simulink library "DQN_Lib (conflicted copy 2023-11-25 155310)"  (R2023b)
settings: Solver=VariableStepAuto  StartTime=0.0  StopTime=10.0  RelTol=1e-3
undefined symbols (not defined in the file): FreqRad, HrmOrd, Init, La, N, R, Ra, TimeStep, Ts, Ts_dqn, Ws
libraries: $bdroot x4, spsMeanVariableFrequencyLib x4, eeTransforms x3, spsabctodq0Lib x2, spsAlphaBetaZerotodq0Lib x1
(part 4 of 8)

== matlab function DQN_Lib (conflicted copy 2023-11-25 155310)/DQn (Full)10 ==
  data: Zdc output size=3; Xdc input size=3; Xdp input; Xdn input; Xdz input; Xqp input; Xqn input; Xqz input; Ydc input size=3; Ydp input; Ydn input; Ydz input; Yqp input; Yqn input; Yqz input; Zdp output; Zdn output; Zdz output; Zqp output; Zqn output; N parameter; Zqz output
function [Zdc,Zdp,Zdn,Zdz,Zqp,Zqn,Zqz]  = MultDQN(Xdc, Xdp, Xdn, Xdz, Xqp, Xqn, Xqz, Ydc, Ydp, Ydn, Ydz, Yqp, Yqn, Yqz, N)

    Zdc = zeros(3,1);
    a = -0.5+0.866i;
    a2 = -0.5-0.866i;
    T = [1 1 1;1 a a2;1 a2 a];

    Xdp = [Xdp; zeros(N-numel(Xdp),1)];
    Ydp = [Ydp; zeros(N-numel(Ydp),1)];
    Xqp = [Xqp; zeros(N-numel(Xqp),1)];
    Yqp = [Yqp; zeros(N-numel(Yqp),1)];
      
    Xdn = [Xdn; zeros(N-numel(Xdn),1)];
    Ydn = [Ydn; zeros(N-numel(Ydn),1)];
    Xqn = [Xqn; zeros(N-numel(Xqn),1)];
    Yqn = [Yqn; zeros(N-numel(Yqn),1)];
    
    Xdz = [Xdz; zeros(N-numel(Xdz),1)];
    Ydz = [Ydz; zeros(N-numel(Ydz),1)];
    Xqz = [Xqz; zeros(N-numel(Xqz),1)];
    Yqz = [Yqz; zeros(N-numel(Yqz),1)];
    
    Zdp = zeros(2*N,1);
    Zdn = zeros(2*N,1);
    Zqp = zeros(2*N,1);
    Zqn = zeros(2*N,1);
    Zdz = zeros(2*N,1);
    Zqz = zeros(2*N,1);
         
    Zdc = Xdc.*Ydc;
    
   
    for h = 1 : 2*N
        if(h<=N)

            Zdc = Zdc + 0.5*(Xdp(h)*Ydp(h)+Xqp(h)*Yqp(h));
            Zdc = Zdc + 0.5*(Xdn(h)*Ydn(h)+Xqn(h)*Yqn(h));
            Zdc = Zdc + 0.5*(Xdz(h)*Ydz(h)+Xqz(h)*Yqz(h));


            Ymp = sqrt(Ydp(h)^2+Yqp(h)^2);
            Yap = atan2(Yqp(h),+Ydp(h));  


            Ymn = sqrt(Ydn(h)^2+Yqn(h)^2);
            Yan = atan2(Yqn(h),-Ydn(h));  

            Xmz = sqrt(Xdz(h)^2+Xqz(h)^2);
            Xaz = atan2(Xqz(h),+Xdz(h));  
            Ymz = sqrt(Ydz(h)^2+Yqz(h)^2);
            Yaz = atan2(Yqz(h),+Ydz(h));  

            
            Xmp = sqrt(Xdp(h)^2+Xqp(h)^2);
            Xap = atan2(Xqp(h),+Xdp(h));  
            if(Xmp~=0)
            Zdz(2*h) = Zdz(2*h) + 0.5*Xmp*Ymn*sin(Xap+Yan);
            Zqz(2*h) = Zqz(2*h) - 0.5*Xmp*Ymn*cos(Xap+Yan);
            Zdc = Zdc + 0.5*Xmp*Ymn*[cos(Xap-Yan); cos(Xap-Yan-4*pi/3); cos(Xap-Yan+4*pi/3)];
            Zdc = Zdc + 0.5*Xmp*Ymz*[cos(Xap-Yaz); cos(Xap-Yaz+4*pi/3); cos(Xap-Yaz-4*pi/3)];
            end

            Xmn = sqrt(Xdn(h)^2+Xqn(h)^2);
            Xan = atan2(Xqn(h),-Xdn(h));  
            if(Xmn~=0)
            Zdz(2*h) = Zdz(2*h) + 0.5*Xmn*Ymp*sin(Xan+Yap);
            Zqz(2*h) = Zqz(2*h) - 0.5*Xmn*Ymp*cos(Xan+Yap);
            Zdc = Zdc + 0.5*Xmn*Ymp*[cos(Xan-Yap); cos(Xan-Yap+4*pi/3); cos(Xan-Yap-4*pi/3)];
            Zdc = Zdc + 0.5*Xmn*Ymz*[cos(Xan-Yaz); cos(Xan-Yaz-4*pi/3); cos(Xan-Yaz+4*pi/3)];
            end
            
            if(Xmz~=0)
            Zdc = Zdc + 0.5*Xmz*Ymp*[cos(Xaz-Yap); cos(Xaz-Yap-4*pi/3); cos(Xaz-Yap+4*pi/3)];
            Zdc = Zdc + 0.5*Xmz*Ymn*[cos(Xaz-Yan); cos(Xaz-Yan+4*pi/3); cos(Xaz-Yan-4*pi/3)];
            end

            if(all(Xdc == Xdc(1)) && all(Ydc == Ydc(1)))
                Zdp(h) = Zdp(h) + Xdc(1)*Ydp(h)+Xdp(h)*Ydc(1);     
                Zqp(h) = Zqp(h) + Xdc(1)*Yqp(h)+Xqp(h)*Ydc(1);  
                Zdn(h) = Zdn(h) + Xdc(1)*Ydn(h)+Xdn(h)*Ydc(1);
                Zqn(h) = Zqn(h) + Xdc(1)*Yqn(h)+Xqn(h)*Ydc(1);
                Zdz(h) = Zdz(h) + Xdc(1)*Ydz(h)+Xdz(h)*Ydc(1);     
                Zqz(h) = Zqz(h) + Xdc(1)*Yqz(h)+Xqz(h)*Ydc(1); 
            else
                %%%%%%%%%%%%%%%%% POSITIVE (Ydc*Xp) %%%%%%%%%%%%%%%%%%%
                if(Xmp ~= 0)
%                     V_ABC = [Ydc(1)*Xmp*(cos(Xap)       +1i*sin(Xap));
%                              Ydc(2)*Xmp*(cos(Xap-2*pi/3)+1i*sin(Xap-2*pi/3));
%                              Ydc(3)*Xmp*(cos(Xap+2*pi/3)+1i*sin(Xap+2*pi/3))];
%                     V_012 = T*V_ABC/3;
                    
                    V_012 = T*[Ydc(1)*Xmp*(cos(Xap)       +1i*sin(Xap));
                               Ydc(2)*Xmp*(cos(Xap-2*pi/3)+1i*sin(Xap-2*pi/3));
                               Ydc(3)*Xmp*(cos(Xap+2*pi/3)+1i*sin(Xap+2*pi/3))]/3;

                    Zdz(h) = Zdz(h) + real(V_012(1)); Zqz(h) = Zqz(h) + imag(V_012(1));
                    Zdp(h) = Zdp(h) + real(V_012(2)); Zqp(h) = Zqp(h) + imag(V_012(2));
                    Zdn(h) = Zdn(h) - real(V_012(3)); Zqn(h) = Zqn(h) + imag(V_012(3));
                end
                %%%%%%%%%%%%%%%%% POSITIVE (Xdc*Yp) %%%%%%%%%%%%%%%%%%%
                if(Ymp ~= 0)
%                 V_ABC = [Xdc(1)*Ymp*(cos(Yap)       +1i*sin(Yap));
%                          Xdc(2)*Ymp*(cos(Yap-2*pi/3)+1i*sin(Yap-2*pi/3));
%                          Xdc(3)*Ymp*(cos(Yap+2*pi/3)+1i*sin(Yap+2*pi/3))];
%                 V_012 = T*V_ABC/3;
                
                V_012 = T*[Xdc(1)*Ymp*(cos(Yap)       +1i*sin(Yap));
                         Xdc(2)*Ymp*(cos(Yap-2*pi/3)+1i*sin(Yap-2*pi/3));
                         Xdc(3)*Ymp*(cos(Yap+2*pi/3)+1i*sin(Yap+2*pi/3))]/3;

                Zdz(h) = Zdz(h) + real(V_012(1)); Zqz(h) = Zqz(h) + imag(V_012(1));
                Zdp(h) = Zdp(h) + real(V_012(2)); Zqp(h) = Zqp(h) + imag(V_012(2));
                Zdn(h) = Zdn(h) - real(V_012(3)); Zqn(h) = Zqn(h) + imag(V_012(3));
                end
                %%%%%%%%%%%%%%%%% NEGATIVE (Ydc*Xn) %%%%%%%%%%%%%%%%%%%
                if(Xmn ~= 0)
                    V_012 = T*[Ydc(1)*Xmn*(cos(Xan)       +1i*sin(Xan));
                             Ydc(2)*Xmn*(cos(Xan+2*pi/3)+1i*sin(Xan+2*pi/3));
                             Ydc(3)*Xmn*(cos(Xan-2*pi/3)+1i*sin(Xan-2*pi/3))]/3;
                    

                    Zdz(h) = Zdz(h) + real(V_012(1)); Zqz(h) = Zqz(h) + imag(V_012(1));
                    Zdp(h) = Zdp(h) + real(V_012(2)); Zqp(h) = Zqp(h) + imag(V_012(2));
                    Zdn(h) = Zdn(h) - real(V_012(3)); Zqn(h) = Zqn(h) + imag(V_012(3));
                end
                %%%%%%%%%%%%%%%%% NEGATIVE (Xdc*Yn) %%%%%%%%%%%%%%%%%%%
                if(Ymn ~= 0)
                    V_012 = T*[Xdc(1)*Ymn*(cos(Yan)       +1i*sin(Yan));
                             Xdc(2)*Ymn*(cos(Yan+2*pi/3)+1i*sin(Yan+2*pi/3));
                             Xdc(3)*Ymn*(cos(Yan-2*pi/3)+1i*sin(Yan-2*pi/3))]/3;

                    Zdz(h) = Zdz(h) + real(V_012(1)); Zqz(h) = Zqz(h) + imag(V_012(1));
                    Zdp(h) = Zdp(h) + real(V_012(2)); Zqp(h) = Zqp(h) + imag(V_012(2));
                    Zdn(h) = Zdn(h) - real(V_012(3)); Zqn(h) = Zqn(h) + imag(V_012(3));
                end
                %%%%%%%%%%%%%%%%%%%%%%%%%%%%%%%%%%%%%%%%%%%%%%%%%%%%%%
                if(Xmz ~= 0)
                    V_012 = T*[Ydc(1)*Xmz*(cos(Xaz)+1i*sin(Xaz));
                               Ydc(2)*Xmz*(cos(Xaz)+1i*sin(Xaz));
                               Ydc(3)*Xmz*(cos(Xaz)+1i*sin(Xaz))]/3;
                    

                    Zdz(h) = Zdz(h) + real(V_012(1)); Zqz(h) = Zqz(h) + imag(V_012(1));
                    Zdp(h) = Zdp(h) + real(V_012(2)); Zqp(h) = Zqp(h) + imag(V_012(2));
                    Zdn(h) = Zdn(h) - real(V_012(3)); Zqn(h) = Zqn(h) + imag(V_012(3));
                end
                %%%%%%%%%%%%%%%%%%%%%%%%%%%%%%%%%%%%%%%%%%%%%%%%%%%%%%

                if(Ymz ~= 0)
                    V_012 = T*[Xdc(1)*Ymz*(cos(Yaz)+1i*sin(Yaz));
                             Xdc(2)*Ymz*(cos(Yaz)+1i*sin(Yaz));
                             Xdc(3)*Ymz*(cos(Yaz)+1i*sin(Yaz))]/3;
                    
                    Zdz(h) = Zdz(h) + real(V_012(1)); Zqz(h) = Zqz(h) + imag(V_012(1));
                    Zdp(h) = Zdp(h) + real(V_012(2)); Zqp(h) = Zqp(h) + imag(V_012(2));
                    Zdn(h) = Zdn(h) - real(V_012(3)); Zqn(h) = Zqn(h) + imag(V_012(3));
                end
            end
            
%%%%%%%%%%%%%%%%%%%%%% h<=N ODD %%%%%%%%%%%%%%%%%%%%%%%%%%%%%%%%%%%%%%%%%
            if(mod(h,2)==1) 
                %%%%%%%%%%%%%%%%% D3p (3ph+) %%%%%%%%%%%%%%%%%%%%%%%

                %&%%%%%%%%%%%%%%%%%%%%%%%%%% PP + NN %%%%%%%%%%%%%%%%%%%%%%%%%%%
                for i = 1 : h - 1
                   Zdp(h) = Zdp(h) - 0.5*(Xdn(i)*Yqn(h-i) + Xqn(i)*Ydn(h-i));                    
                   Zdn(h) = Zdn(h) - 0.5*(Xdp(i)*Yqp(h-i) + Xqp(i)*Ydp(h-i)); 
                   Zqp(h) = Zqp(h) - 0.5*(Xdn(i)*Ydn(h-i) - Xqn(i)*Yqn(h-i));                
                   Zqn(h) = Zqn(h) - 0.5*(Xdp(i)*Ydp(h-i) - Xqp(i)*Yqp(h-i)); 
                end

                for i = 1 : N - h
                    Zdz(h) = Zdz(h) + 0.5*(-Xdp(i)*Yqp(i+h) + Xqp(i)*Ydp(i+h) + Xdp(i+h)*Yqp(i) - Xqp(i+h)*Ydp(i) + Xdn(i)*Yqn(i+h) - Xqn(i)*Ydn(i+h) - Xdn(i+h)*Yqn(i) + Xqn(i+h)*Ydn(i));  
                    Zqz(h) = Zqz(h) + 0.5*(+Xdp(i)*Ydp(i+h) + Xqp(i)*Yqp(i+h) + Xdp(i+h)*Ydp(i) + Xqp(i+h)*Yqp(i) + Xdn(i)*Ydn(i+h) + Xqn(i)*Yqn(i+h) + Xdn(i+h)*Ydn(i) + Xqn(i+h)*Yqn(i));    
                end
                %&%%%%%%%%%%%%%%%%%%%%%%%%%% PP + NN %%%%%%%%%%%%%%%%%%%%%%%%%%%

                for k = 1 : (N + mod(N+1,2) - h)/2
                    i = 2*k-1;
                    j = i+h;

                    Zdz(h)  = Zdz(h)  + 0.5*(-Xdz(i)*Yqz(j) + Xqz(i)*Ydz(j) + Xdz(j)*Yqz(i) - Xqz(j)*Ydz(i));
                    Zqz(h)  = Zqz(h)  + 0.5*(+Xdz(i)*Ydz(j) + Xqz(i)*Yqz(j) + Xdz(j)*Ydz(i) + Xqz(j)*Yqz(i)); 

                    Zdp(h) = Zdp(h) + 0.5*(-Xdp(i)*Yqn(j) - Xqp(i)*Ydn(j) - Xdn(j)*Yqp(i) - Xqn(j)*Ydp(i)); 
                    Zdp(h) = Zdp(h) + 0.5*(-Xdz(i)*Yqp(j) + Xqz(i)*Ydp(j) + Xdp(j)*Yqz(i) - Xqp(j)*Ydz(i));    
                    Zdp(h) = Zdp(h) + 0.5*(+Xdn(i)*Yqz(j) + Xqn(i)*Ydz(j) + Xdz(j)*Yqn(i) + Xqz(j)*Ydn(i));
                    
                    Zqp(h) = Zqp(h) + 0.5*(-Xdp(i)*Ydn(j) + Xqp(i)*Yqn(j) - Xdn(j)*Ydp(i) + Xqn(j)*Yqp(i));  
                    Zqp(h) = Zqp(h) + 0.5*(+Xdz(i)*Ydp(j) + Xqz(i)*Yqp(j) + Xdp(j)*Ydz(i) + Xqp(j)*Yqz(i));     
                    Zqp(h) = Zqp(h) + 0.5*(-Xdn(i)*Ydz(j) + Xqn(i)*Yqz(j) - Xdz(j)*Ydn(i) + Xqz(j)*Yqn(i));

                    Zdn(h) = Zdn(h) + 0.5*(+Xdp(i)*Yqz(j) - Xqp(i)*Ydz(j) - Xdz(j)*Yqp(i) + Xqz(j)*Ydp(i));             
                    Zdn(h) = Zdn(h) + 0.5*(+Xdz(i)*Yqn(j) + Xqz(i)*Ydn(j) + Xdn(j)*Yqz(i) + Xqn(j)*Ydz(i));
                    Zdn(h) = Zdn(h) + 0.5*(-Xdn(i)*Yqp(j) - Xqn(i)*Ydp(j) - Xdp(j)*Yqn(i) - Xqp(j)*Ydn(i)); 

                    Zqn(h) = Zqn(h) + 0.5*(+Xdp(i)*Ydz(j) + Xqp(i)*Yqz(j) + Xdz(j)*Ydp(i) + Xqz(j)*Yqp(i)); 
                    Zqn(h) = Zqn(h) + 0.5*(-Xdz(i)*Ydn(j) + Xqz(i)*Yqn(j) - Xdn(j)*Ydz(i) + Xqn(j)*Yqz(i)); 
                    Zqn(h) = Zqn(h) + 0.5*(-Xdn(i)*Ydp(j) + Xqn(i)*Yqp(j) - Xdp(j)*Ydn(i) + Xqp(j)*Yqn(i));  
                end

                for k = 1 : (N + mod(N,2) - h - 1)/2
                    i = 2*k;
                    j = i+h;
                    
                    Zdz(h) = Zdz(h)   + 0.5*(-Xdz(i)*Yqz(j) + Xqz(i)*Ydz(j) + Xdz(j)*Yqz(i) - Xqz(j)*Ydz(i));
                    Zqz(h) = Zqz(h)   + 0.5*(+Xdz(i)*Ydz(j) + Xqz(i)*Yqz(j) + Xdz(j)*Ydz(i) + Xqz(j)*Yqz(i)); 

                    Zdp(h) = Zdp(h) + 0.5*(-Xdp(i)*Yqn(j) - Xqp(i)*Ydn(j) - Xdn(j)*Yqp(i) - Xqn(j)*Ydp(i)); 
                    Zqp(h) = Zqp(h) + 0.5*(-Xdp(i)*Ydn(j) + Xqp(i)*Yqn(j) - Xdn(j)*Ydp(i) + Xqn(j)*Yqp(i));  
                    Zdn(h) = Zdn(h) + 0.5*(-Xdn(i)*Yqp(j) - Xqn(i)*Ydp(j) - Xdp(j)*Yqn(i) - Xqp(j)*Ydn(i)); 
                    Zqn(h) = Zqn(h) + 0.5*(-Xdn(i)*Ydp(j) + Xqn(i)*Yqp(j) - Xdp(j)*Ydn(i) + Xqp(j)*Yqn(i));                                          

                    Zdp(h) = Zdp(h) + 0.5*(-Xdz(i)*Yqp(j) + Xqz(i)*Ydp(j) + Xdp(j)*Yqz(i) - Xqp(j)*Ydz(i));
                    Zqp(h) = Zqp(h) + 0.5*(+Xdz(i)*Ydp(j) + Xqz(i)*Yqp(j) + Xdp(j)*Ydz(i) + Xqp(j)*Yqz(i));                     
                    Zdn(h) = Zdn(h) + 0.5*(+Xdp(i)*Yqz(j) - Xqp(i)*Ydz(j) - Xdz(j)*Yqp(i) + Xqz(j)*Ydp(i));
                    Zqn(h) = Zqn(h) + 0.5*(+Xdp(i)*Ydz(j) + Xqp(i)*Yqz(j) + Xdz(j)*Ydp(i) + Xqz(j)*Yqp(i));   

                    Zdp(h) = Zdp(h) + 0.5*(+Xdn(i)*Yqz(j) + Xqn(i)*Ydz(j) + Xdz(j)*Yqn(i) + Xqz(j)*Ydn(i));
                    Zqp(h) = Zqp(h) + 0.5*(-Xdn(i)*Ydz(j) + Xqn(i)*Yqz(j) - Xdz(j)*Ydn(i) + Xqz(j)*Yqn(i));                
                    Zdn(h) = Zdn(h) + 0.5*(+Xdz(i)*Yqn(j) + Xqz(i)*Ydn(j) + Xdn(j)*Yqz(i) + Xqn(j)*Ydz(i));
                    Zqn(h) = Zqn(h) + 0.5*(-Xdz(i)*Ydn(j) + Xqz(i)*Yqn(j) - Xdn(j)*Ydz(i) + Xqn(j)*Yqz(i)); 

                end

                for k = (h-1)/2:-1:1
                    i = k;
                    j = h-i;  
                    
                    Zdz(h) = Zdz(h) + 0.5*(+Xdp(i)*Yqn(j)-Xqp(i)*Ydn(j)-Xdn(j)*Yqp(i)+Xqn(j)*Ydp(i));
                    Zqz(h) = Zqz(h) + 0.5*(+Xdp(i)*Ydn(j)+Xqp(i)*Yqn(j)+Xdn(j)*Ydp(i)+Xqn(j)*Yqp(i));
                    Zdz(h) = Zdz(h) + 0.5*(+Xdp(j)*Yqn(i)-Xqp(j)*Ydn(i)-Xdn(i)*Yqp(j)+Xqn(i)*Ydp(j));
                    Zqz(h) = Zqz(h) + 0.5*(+Xdp(j)*Ydn(i)+Xqp(j)*Yqn(i)+Xdn(i)*Ydp(j)+Xqn(i)*Yqp(j)); 
                    Zdz(h) = Zdz(h) + 0.5*(+Xdz(i)*Yqz(j)+Xqz(i)*Ydz(j)+Xdz(j)*Yqz(i)+Xqz(j)*Ydz(i));
                    Zqz(h) = Zqz(h) + 0.5*(-Xdz(i)*Ydz(j)+Xqz(i)*Yqz(j)-Xdz(j)*Ydz(i)+Xqz(j)*Yqz(i));    
                        
                        
                    Zdp(h) = Zdp(h) + 0.5*(+Xdz(i)*Yqp(j)+Xqz(i)*Ydp(j)+Xdz(j)*Yqp(i)+Xqz(j)*Ydp(i));
                    Zqp(h) = Zqp(h) + 0.5*(-Xdz(i)*Ydp(j)+Xqz(i)*Yqp(j)-Xdz(j)*Ydp(i)+Xqz(j)*Yqp(i));
                    Zdp(h) = Zdp(h) + 0.5*(+Xdp(i)*Yqz(j)+Xqp(i)*Ydz(j)+Xdp(j)*Yqz(i)+Xqp(j)*Ydz(i));
                    Zqp(h) = Zqp(h) + 0.5*(-Xdp(i)*Ydz(j)+Xqp(i)*Yqz(j)-Xdp(j)*Ydz(i)+Xqp(j)*Yqz(i)); 
                    
                              
                    Zdn(h) = Zdn(h) + 0.5*(+Xdn(i)*Yqz(j)-Xqn(i)*Ydz(j)+Xdn(j)*Yqz(i)-Xqn(j)*Ydz(i));
                    Zqn(h) = Zqn(h) + 0.5*(+Xdn(i)*Ydz(j)+Xqn(i)*Yqz(j)+Xdn(j)*Ydz(i)+Xqn(j)*Yqz(i)); 
                    Zdn(h) = Zdn(h) + 0.5*(-Xdz(i)*Yqn(j)+Xqz(i)*Ydn(j)-Xdz(j)*Yqn(i)+Xqz(j)*Ydn(i));
                    Zqn(h) = Zqn(h) + 0.5*(+Xdz(i)*Ydn(j)+Xqz(i)*Yqn(j)+Xdz(j)*Ydn(i)+Xqz(j)*Yqn(i)); 
                end
%%%%%%%%%%%%%%%%%%%%%% h<=N EVEN %%%%%%%%%%%%%%%%%%%%%%%%%%%%%%%%%%%%%%%%%           
            else 
               
                Zdp(h) = Zdp(h) + 0.5*(-Xdn(h/2)*Yqn(h/2)-Xqn(h/2)*Ydn(h/2));   
                Zqp(h) = Zqp(h) + 0.5*(-Xdn(h/2)*Ydn(h/2)+Xqn(h/2)*Yqn(h/2)); 
                Zdn(h) = Zdn(h) + 0.5*(-Xdp(h/2)*Yqp(h/2)-Xqp(h/2)*Ydp(h/2));   
                Zqn(h) = Zqn(h) + 0.5*(-Xdp(h/2)*Ydp(h/2)+Xqp(h/2)*Yqp(h/2));   

                Zdz(h)  = Zdz(h)  + 0.5*(+Xdz(h/2)*Yqz(h/2)+Xqz(h/2)*Ydz(h/2));
                Zqz(h)  = Zqz(h)  + 0.5*(-Xdz(h/2)*Ydz(h/2)+Xqz(h/2)*Yqz(h/2));

                Zdp(h) = Zdp(h) + 0.5*(+Xdz(h/2)*Yqp(h/2)+Xqz(h/2)*Ydp(h/2)+Xdp(h/2)*Yqz(h/2)+Xqp(h/2)*Ydz(h/2));   
                Zqp(h) = Zqp(h) + 0.5*(-Xdz(h/2)*Ydp(h/2)+Xqz(h/2)*Yqp(h/2)-Xdp(h/2)*Ydz(h/2)+Xqp(h/2)*Yqz(h/2)); 
                Zdn(h) = Zdn(h) + 0.5*(+Xdn(h/2)*Yqz(h/2)-Xqn(h/2)*Ydz(h/2)-Xdz(h/2)*Yqn(h/2)+Xqz(h/2)*Ydn(h/2));   
                Zqn(h) = Zqn(h) + 0.5*(+Xdn(h/2)*Ydz(h/2)+Xqn(h/2)*Yqz(h/2)+Xdz(h/2)*Ydn(h/2)+Xqz(h/2)*Yqn(h/2));    
                
                for k = 1:N-h
                    i = k;
                    j = h+i;
                
                    Zdz(h) = Zdz(h)   + 0.5*(+Xdp(j)*Yqp(i) - Xqp(j)*Ydp(i) - Xdp(i)*Yqp(j) + Xqp(i)*Ydp(j));
                    Zqz(h) = Zqz(h)   + 0.5*(+Xdp(j)*Ydp(i) + Xqp(j)*Yqp(i) + Xdp(i)*Ydp(j) + Xqp(i)*Yqp(j));                                           
                    Zdz(h) = Zdz(h)   + 0.5*(+Xdn(i)*Yqn(j) - Xqn(i)*Ydn(j) - Xdn(j)*Yqn(i) + Xqn(j)*Ydn(i));
                    Zqz(h) = Zqz(h)   + 0.5*(+Xdn(i)*Ydn(j) + Xqn(i)*Yqn(j) + Xdn(j)*Ydn(i) + Xqn(j)*Yqn(i));  
                    Zdz(h) = Zdz(h)   + 0.5*(-Xdz(i)*Yqz(j) + Xqz(i)*Ydz(j) + Xdz(j)*Yqz(i) - Xqz(j)*Ydz(i));
                    Zqz(h) = Zqz(h)   + 0.5*(+Xdz(i)*Ydz(j) + Xqz(i)*Yqz(j) + Xdz(j)*Ydz(i) + Xqz(j)*Yqz(i)); 
                                       
                    Zdp(h) = Zdp(h) + 0.5*(-Xdp(i)*Yqn(j) - Xqp(i)*Ydn(j) - Xdn(j)*Yqp(i) - Xqn(j)*Ydp(i)); 
                    Zqp(h) = Zqp(h) + 0.5*(-Xdp(i)*Ydn(j) + Xqp(i)*Yqn(j) - Xdn(j)*Ydp(i) + Xqn(j)*Yqp(i)); 
                    Zdn(h) = Zdn(h) + 0.5*(-Xdn(i)*Yqp(j) - Xqn(i)*Ydp(j) - Xdp(j)*Yqn(i) - Xqp(j)*Ydn(i)); 
                    Zqn(h) = Zqn(h) + 0.5*(-Xdn(i)*Ydp(j) + Xqn(i)*Yqp(j) - Xdp(j)*Ydn(i) + Xqp(j)*Yqn(i)); 
                        
                    Zdp(h) = Zdp(h) + 0.5*(+Xdp(j)*Yqz(i) - Xqp(j)*Ydz(i) - Xdz(i)*Yqp(j) + Xqz(i)*Ydp(j));
                    Zqp(h) = Zqp(h) + 0.5*(+Xdp(j)*Ydz(i) + Xqp(j)*Yqz(i) + Xdz(i)*Ydp(j) + Xqz(i)*Yqp(j)); 
                    Zdn(h) = Zdn(h) + 0.5*(+Xdp(i)*Yqz(j) - Xqp(i)*Ydz(j) - Xdz(j)*Yqp(i) + Xqz(j)*Ydp(i));
                    Zqn(h) = Zqn(h) + 0.5*(+Xdp(i)*Ydz(j) + Xqp(i)*Yqz(j) + Xdz(j)*Ydp(i) + Xqz(j)*Yqp(i)); 
                    
                    Zdp(h) = Zdp(h) + 0.5*(+Xdn(i)*Yqz(j) + Xqn(i)*Ydz(j) + Xdz(j)*Yqn(i) + Xqz(j)*Ydn(i));
                    Zqp(h) = Zqp(h) + 0.5*(-Xdn(i)*Ydz(j) + Xqn(i)*Yqz(j) - Xdz(j)*Ydn(i) + Xqz(j)*Yqn(i)); 
                    Zdn(h) = Zdn(h) + 0.5*(+Xdn(j)*Yqz(i) + Xqn(j)*Ydz(i) + Xdz(i)*Yqn(j) + Xqz(i)*Ydn(j));
                    Zqn(h) = Zqn(h) + 0.5*(-Xdn(j)*Ydz(i) + Xqn(j)*Yqz(i) - Xdz(i)*Ydn(j) + Xqz(i)*Yqn(j)); 
                end

                for k = h/2-1:-1:1
                    i = k;
                    j = h-i;   

                    Zdz(h) = Zdz(h)   + 0.5*(+Xdp(i)*Yqn(j) - Xqp(i)*Ydn(j) + Xdp(j)*Yqn(i) - Xqp(j)*Ydn(i));
                    Zdz(h) = Zdz(h)   + 0.5*(-Xdn(i)*Yqp(j) + Xqn(i)*Ydp(j) - Xdn(j)*Yqp(i) + Xqn(j)*Ydp(i));      
                    Zdz(h) = Zdz(h)   + 0.5*(+Xdz(i)*Yqz(j) + Xqz(i)*Ydz(j) + Xdz(j)*Yqz(i) + Xqz(j)*Ydz(i));
                    
                    Zqz(h) = Zqz(h)   + 0.5*(+Xdp(i)*Ydn(j) + Xqp(i)*Yqn(j) + Xdp(j)*Ydn(i) + Xqp(j)*Yqn(i)); 
                    Zqz(h) = Zqz(h)   + 0.5*(+Xdn(i)*Ydp(j) + Xqn(i)*Yqp(j) + Xdn(j)*Ydp(i) + Xqn(j)*Yqp(i));
                    Zqz(h) = Zqz(h)   + 0.5*(-Xdz(i)*Ydz(j) + Xqz(i)*Yqz(j) - Xdz(j)*Ydz(i) + Xqz(j)*Yqz(i)); 
                    
                    Zdp(h) = Zdp(h) + 0.5*(+Xdp(i)*Yqz(j) + Xqp(i)*Ydz(j) + Xdp(j)*Yqz(i) + Xqp(j)*Ydz(i)); 
                    Zdp(h) = Zdp(h) + 0.5*(-Xdn(i)*Yqn(j) - Xqn(i)*Ydn(j) - Xdn(j)*Yqn(i) - Xqn(j)*Ydn(i)); 
                    Zdp(h) = Zdp(h) + 0.5*(+Xdz(i)*Yqp(j) + Xqz(i)*Ydp(j) + Xdz(j)*Yqp(i) + Xqz(j)*Ydp(i));
                    
                    Zqp(h) = Zqp(h) + 0.5*(-Xdp(i)*Ydz(j) + Xqp(i)*Yqz(j) - Xdp(j)*Ydz(i) + Xqp(j)*Yqz(i)); 
                    Zqp(h) = Zqp(h) + 0.5*(-Xdn(i)*Ydn(j) + Xqn(i)*Yqn(j) - Xdn(j)*Ydn(i) + Xqn(j)*Yqn(i));
                    Zqp(h) = Zqp(h) + 0.5*(-Xdz(i)*Ydp(j) + Xqz(i)*Yqp(j) - Xdz(j)*Ydp(i) + Xqz(j)*Yqp(i));  
                    
                    Zdn(h) = Zdn(h) + 0.5*(-Xdp(i)*Yqp(j) - Xqp(i)*Ydp(j) - Xdp(j)*Yqp(i) - Xqp(j)*Ydp(i));
                    Zdn(h) = Zdn(h) + 0.5*(+Xdn(i)*Yqz(j) - Xqn(i)*Ydz(j) + Xdn(j)*Yqz(i) - Xqn(j)*Ydz(i));
                    Zdn(h) = Zdn(h) + 0.5*(-Xdz(i)*Yqn(j) + Xqz(i)*Ydn(j) - Xdz(j)*Yqn(i) + Xqz(j)*Ydn(i));
                    
                    Zqn(h) = Zqn(h) + 0.5*(-Xdp(i)*Ydp(j) + Xqp(i)*Yqp(j) - Xdp(j)*Ydp(i) + Xqp(j)*Yqp(i));  
                    Zqn(h) = Zqn(h) + 0.5*(+Xdn(i)*Ydz(j) + Xqn(i)*Yqz(j) + Xdn(j)*Ydz(i) + Xqn(j)*Yqz(i));
                    Zqn(h) = Zqn(h) + 0.5*(+Xdz(i)*Ydn(j) + Xqz(i)*Yqn(j) + Xdz(j)*Ydn(i) + Xqz(j)*Yqn(i)); 
                end
            end
%%%%%%%%%%%%%%%%%%%%%%%%%%%% h>N  %%%%%%%%%%%%%%%%%%%%%%%%%%%%%%%%%%%%%%%%% 
        else %h>N
            
            
            %%%%%%%%%%%%%%%%%%%%%%%%%%% PP + NN %%%%%%%%%%%%%%%%%%%%%%%%%%%
            for i = h-N : N
                Zdp(h) = Zdp(h) - 0.5*(Xdn(i)*Yqn(h-i) + Xqn(i)*Ydn(h-i));                
                Zdn(h) = Zdn(h) - 0.5*(Xdp(i)*Yqp(h-i) + Xqp(i)*Ydp(h-i));                     
                Zqp(h) = Zqp(h) - 0.5*(Xdn(i)*Ydn(h-i) - Xqn(i)*Yqn(h-i));                      
                Zqn(h) = Zqn(h) - 0.5*(Xdp(i)*Ydp(h-i) - Xqp(i)*Yqp(h-i));   
            end
            %%%%%%%%%%%%%%%%%%%%%%%%%%% PP + NN %%%%%%%%%%%%%%%%%%%%%%%%%%%

            if(mod(h,2)==1) %%%%%%%%%%% h>N ODD %%%%%%%%%%%%%%%%%%%

                for k = (h-1)/2:-1:h-N
                    i = k;
                    j = h-i;
                    
                    Zdz(h) = Zdz(h) + 0.5*(+Xdp(i)*Yqn(j)-Xqp(i)*Ydn(j)-Xdn(j)*Yqp(i)+Xqn(j)*Ydp(i));                  
                    Zdz(h) = Zdz(h) + 0.5*(+Xdp(j)*Yqn(i)-Xqp(j)*Ydn(i)-Xdn(i)*Yqp(j)+Xqn(i)*Ydp(j));
                    Zdz(h) = Zdz(h) + 0.5*(+Xdz(i)*Yqz(j)+Xqz(i)*Ydz(j)+Xdz(j)*Yqz(i)+Xqz(j)*Ydz(i));
                    
                    Zqz(h) = Zqz(h) + 0.5*(-Xdz(i)*Ydz(j)+Xqz(i)*Yqz(j)-Xdz(j)*Ydz(i)+Xqz(j)*Yqz(i));
                    Zqz(h) = Zqz(h) + 0.5*(+Xdp(i)*Ydn(j)+Xqp(i)*Yqn(j)+Xdn(j)*Ydp(i)+Xqn(j)*Yqp(i));
                    Zqz(h) = Zqz(h) + 0.5*(+Xdp(j)*Ydn(i)+Xqp(j)*Yqn(i)+Xdn(i)*Ydp(j)+Xqn(i)*Yqp(j));  
                    
                    Zdp(h) = Zdp(h) + 0.5*(+Xdp(i)*Yqz(j)+Xqp(i)*Ydz(j)+Xdp(j)*Yqz(i)+Xqp(j)*Ydz(i));
                    Zdp(h) = Zdp(h) + 0.5*(+Xdz(i)*Yqp(j)+Xqz(i)*Ydp(j)+Xdz(j)*Yqp(i)+Xqz(j)*Ydp(i));
                    
                    Zqp(h) = Zqp(h) + 0.5*(-Xdp(i)*Ydz(j)+Xqp(i)*Yqz(j)-Xdp(j)*Ydz(i)+Xqp(j)*Yqz(i)); 
                    Zqp(h) = Zqp(h) + 0.5*(-Xdz(i)*Ydp(j)+Xqz(i)*Yqp(j)-Xdz(j)*Ydp(i)+Xqz(j)*Yqp(i));     
                                       
                    Zdn(h) = Zdn(h) + 0.5*(+Xdn(i)*Yqz(j)-Xqn(i)*Ydz(j)+Xdn(j)*Yqz(i)-Xqn(j)*Ydz(i));
                    Zdn(h) = Zdn(h) + 0.5*(-Xdz(i)*Yqn(j)+Xqz(i)*Ydn(j)-Xdz(j)*Yqn(i)+Xqz(j)*Ydn(i));
                    
                    Zqn(h) = Zqn(h) + 0.5*(+Xdn(i)*Ydz(j)+Xqn(i)*Yqz(j)+Xdn(j)*Ydz(i)+Xqn(j)*Yqz(i));
                    Zqn(h) = Zqn(h) + 0.5*(+Xdz(i)*Ydn(j)+Xqz(i)*Yqn(j)+Xdz(j)*Ydn(i)+Xqz(j)*Yqn(i));    

                end

            else %%%%%%%%%%% h>N EVEN %%%%%%%%%%%%%%%%%%%

                Zdz(h)  = Zdz(h)  + 0.5*(+Xdz(h/2)*Yqz(h/2)+Xqz(h/2)*Ydz(h/2));
                Zqz(h)  = Zqz(h)  + 0.5*(-Xdz(h/2)*Ydz(h/2)+Xqz(h/2)*Yqz(h/2));
                
                Zdp(h) = 0.5*(-Xdn(h/2)*Yqn(h/2)-Xqn(h/2)*Ydn(h/2));          
                Zdp(h) = Zdp(h) + 0.5*(+Xdp(h/2)*Yqz(h/2)+Xqp(h/2)*Ydz(h/2));                
                Zdp(h) = Zdp(h) + 0.5*(+Xdz(h/2)*Yqp(h/2)+Xqz(h/2)*Ydp(h/2));    
                
                Zqp(h) = 0.5*(-Xdn(h/2)*Ydn(h/2)+Xqn(h/2)*Yqn(h/2));             
                Zqp(h) = Zqp(h) + 0.5*(-Xdp(h/2)*Ydz(h/2)+Xqp(h/2)*Yqz(h/2));        
                Zqp(h) = Zqp(h) + 0.5*(-Xdz(h/2)*Ydp(h/2)+Xqz(h/2)*Yqp(h/2)); 
                
                Zdn(h) = 0.5*(-Xdp(h/2)*Yqp(h/2)-Xqp(h/2)*Ydp(h/2)); 
                Zdn(h) = Zdn(h) + 0.5*(+Xdn(h/2)*Yqz(h/2)-Xqn(h/2)*Ydz(h/2));
                Zdn(h) = Zdn(h) + 0.5*(-Xdz(h/2)*Yqn(h/2)+Xqz(h/2)*Ydn(h/2));
                               
                Zqn(h) = 0.5*(-Xdp(h/2)*Ydp(h/2)+Xqp(h/2)*Yqp(h/2)); 
                Zqn(h) = Zqn(h) + 0.5*(+Xdn(h/2)*Ydz(h/2)+Xqn(h/2)*Yqz(h/2));        
                Zqn(h) = Zqn(h) + 0.5*(+Xdz(h/2)*Ydn(h/2)+Xqz(h/2)*Yqn(h/2)); 

                for i = (h+2)/2:N
                    j = h-i;
                    Zdz(h)  = Zdz(h)  + 0.5*(+Xdp(i)*Yqn(j)-Xqp(i)*Ydn(j)+Xdp(j)*Yqn(i)-Xqp(j)*Ydn(i));
                    Zdz(h)  = Zdz(h)  + 0.5*(-Xdn(i)*Yqp(j)+Xqn(i)*Ydp(j)-Xdn(j)*Yqp(i)+Xqn(j)*Ydp(i));
                    Zdz(h)  = Zdz(h)  + 0.5*(+Xdz(i)*Yqz(j)+Xqz(i)*Ydz(j)+Xdz(j)*Yqz(i)+Xqz(j)*Ydz(i));
                    
                    Zqz(h)  = Zqz(h)  + 0.5*(+Xdp(i)*Ydn(j)+Xqp(i)*Yqn(j)+Xdp(j)*Ydn(i)+Xqp(j)*Yqn(i));                      
                    Zqz(h)  = Zqz(h)  + 0.5*(+Xdn(i)*Ydp(j)+Xqn(i)*Yqp(j)+Xdn(j)*Ydp(i)+Xqn(j)*Yqp(i));  
                    Zqz(h)  = Zqz(h)  + 0.5*(-Xdz(i)*Ydz(j)+Xqz(i)*Yqz(j)-Xdz(j)*Ydz(i)+Xqz(j)*Yqz(i));
                    
                    Zdp(h) = Zdp(h) + 0.5*(+Xdp(i)*Yqz(j)+Xqp(i)*Ydz(j)+Xdp(j)*Yqz(i)+Xqp(j)*Ydz(i));  
                    Zdp(h) = Zdp(h) + 0.5*(-Xdn(i)*Yqn(j)-Xqn(i)*Ydn(j)-Xdn(j)*Yqn(i)-Xqn(j)*Ydn(i));             
                    Zdp(h) = Zdp(h) + 0.5*(+Xdz(i)*Yqp(j)+Xqz(i)*Ydp(j)+Xdz(j)*Yqp(i)+Xqz(j)*Ydp(i));           
                    
                    Zqp(h) = Zqp(h) + 0.5*(-Xdp(i)*Ydz(j)+Xqp(i)*Yqz(j)-Xdp(j)*Ydz(i)+Xqp(j)*Yqz(i));
                    Zqp(h) = Zqp(h) + 0.5*(-Xdn(i)*Ydn(j)+Xqn(i)*Yqn(j)-Xdn(j)*Ydn(i)+Xqn(j)*Yqn(i));    
                    Zqp(h) = Zqp(h) + 0.5*(-Xdz(i)*Ydp(j)+Xqz(i)*Yqp(j)-Xdz(j)*Ydp(i)+Xqz(j)*Yqp(i));   
                    
                    Zdn(h) = Zdn(h) + 0.5*(-Xdp(i)*Yqp(j)-Xqp(i)*Ydp(j)-Xdp(j)*Yqp(i)-Xqp(j)*Ydp(i));
                    Zdn(h) = Zdn(h) + 0.5*(+Xdn(i)*Yqz(j)-Xqn(i)*Ydz(j)+Xdn(j)*Yqz(i)-Xqn(j)*Ydz(i));
                    Zdn(h) = Zdn(h) + 0.5*(-Xdz(i)*Yqn(j)+Xqz(i)*Ydn(j)-Xdz(j)*Yqn(i)+Xqz(j)*Ydn(i));              
                    
                    Zqn(h) = Zqn(h) + 0.5*(-Xdp(i)*Ydp(j)+Xqp(i)*Yqp(j)-Xdp(j)*Ydp(i)+Xqp(j)*Yqp(i));
                    Zqn(h) = Zqn(h) + 0.5*(+Xdn(i)*Ydz(j)+Xqn(i)*Yqz(j)+Xdn(j)*Ydz(i)+Xqn(j)*Yqz(i)); 
                    Zqn(h) = Zqn(h) + 0.5*(+Xdz(i)*Ydn(j)+Xqz(i)*Yqn(j)+Xdz(j)*Ydn(i)+Xqz(j)*Yqn(i));  
                end
            end
        end  
    end
end
  

% function [Zdc,Zdp,Zdn,Zdz,Zqp,Zqn,Zqz]  = MultDQN(Xdc, Xdp, Xdn, Xdz, Xqp, Xqn, Xqz, Ydc, Ydp, Ydn, Ydz, Yqp, Yqn, Yqz, N)
% 
%     Zdc = zeros(3,1);
%     a = -0.5+0.866i;
%     a2 = -0.5-0.866i;
%     T = [1 1 1;1 a a2;1 a2 a];
% 
%     Xdp = [Xdp; zeros(N-numel(Xdp),1)];
%     Ydp = [Ydp; zeros(N-numel(Ydp),1)];
%     Xqp = [Xqp; zeros(N-numel(Xqp),1)];
%     Yqp = [Yqp; zeros(N-numel(Yqp),1)];
%       
%     Xdn = [Xdn; zeros(N-numel(Xdn),1)];
%     Ydn = [Ydn; zeros(N-numel(Ydn),1)];
%     Xqn = [Xqn; zeros(N-numel(Xqn),1)];
%     Yqn = [Yqn; zeros(N-numel(Yqn),1)];
%     
%     Xdz = [Xdz; zeros(N-numel(Xdz),1)];
%     Ydz = [Ydz; zeros(N-numel(Ydz),1)];
%     Xqz = [Xqz; zeros(N-numel(Xqz),1)];
%     Yqz = [Yqz; zeros(N-numel(Yqz),1)];
%        
%     Zdp = zeros(1,2*N);
%     Zdn = zeros(1,2*N);
%     Zqp = zeros(1,2*N);
%     Zqn = zeros(1,2*N);
%     Zdz = zeros(1,2*N);
%     Zqz = zeros(1,2*N);
%    
%     Zdc = Xdc.*Ydc;
%     
%     
%     for h = 1 : N 
% %         Zdc = Zdc + 0.5*(Xdp(h)*Ydp(h)+Xqp(h)*Yqp(h));
% %         Zdc = Zdc + 0.5*(Xdn(h)*Ydn(h)+Xqn(h)*Yqn(h));
% %         Zdc = Zdc + 0.5*(Xdz(h)*Ydz(h)+Xqz(h)*Yqz(h));
% 
%         Xmp = sqrt(Xdp(h)^2+Xqp(h)^2);
%         Xap = atan2(Xqp(h),+Xdp(h));  
%         Ymp = sqrt(Ydp(h)^2+Yqp(h)^2);
%         Yap = atan2(Yqp(h),+Ydp(h));  
% 
%         Xmn = sqrt(Xdn(h)^2+Xqn(h)^2);
%         Xan = atan2(Xqn(h),-Xdn(h));  
%         Ymn = sqrt(Ydn(h)^2+Yqn(h)^2);
%         Yan = atan2(Yqn(h),-Ydn(h));  
% 
%         Xmz = sqrt(Xdz(h)^2+Xqz(h)^2);
%         Xaz = atan2(Xqz(h),+Xdz(h));  
%         Ymz = sqrt(Ydz(h)^2+Yqz(h)^2);
%         Yaz = atan2(Yqz(h),+Ydz(h));  
% 
%         Zdz(2*h) = Zdz(2*h) + 0.5*Xmp*Ymn*sin(Xap+Yan);
%         Zqz(2*h) = Zqz(2*h) - 0.5*Xmp*Ymn*cos(Xap+Yan);
% 
%         Zdz(2*h) = Zdz(2*h) + 0.5*Xmn*Ymp*sin(Xan+Yap);
%         Zqz(2*h) = Zqz(2*h) - 0.5*Xmn*Ymp*cos(Xan+Yap);
% 
% %         Zdc = Zdc + 0.5*Xmp*Ymn*[cos(Xap-Yan) cos(Xap-Yan-4*pi/3) cos(Xap-Yan+4*pi/3)];
% %         Zdc = Zdc + 0.5*Xmn*Ymp*[cos(Xan-Yap) cos(Xan-Yap+4*pi/3) cos(Xan-Yap-4*pi/3)];
% %         Zdc = Zdc + 0.5*Xmz*Ymp*[cos(Xaz-Yap) cos(Xaz-Yap-4*pi/3) cos(Xaz-Yap+4*pi/3)];
% %         Zdc = Zdc + 0.5*Xmp*Ymz*[cos(Xap-Yaz) cos(Xap-Yaz+4*pi/3) cos(Xap-Yaz-4*pi/3)];
% %         Zdc = Zdc + 0.5*Xmn*Ymz*[cos(Xan-Yaz) cos(Xan-Yaz-4*pi/3) cos(Xan-Yaz+4*pi/3)];
% %         Zdc = Zdc + 0.5*Xmz*Ymn*[cos(Xaz-Yan) cos(Xaz-Yan+4*pi/3) cos(Xaz-Yan-4*pi/3)];
% 
%         if(all(Xdc == Xdc(1)) && all(Ydc == Ydc(1)))
%             Zdp(h) = Zdp(h) + Xdc(1)*Ydp(h)+Xdp(h)*Ydc(1);     
%             Zqp(h) = Zqp(h) + Xdc(1)*Yqp(h)+Xqp(h)*Ydc(1);  
%             Zdn(h) = Zdn(h) + Xdc(1)*Ydn(h)+Xdn(h)*Ydc(1);
%             Zqn(h) = Zqn(h) + Xdc(1)*Yqn(h)+Xqn(h)*Ydc(1);
%             Zdz(h) = Zdz(h) + Xdc(1)*Ydz(h)+Xdz(h)*Ydc(1);     
%             Zqz(h) = Zqz(h) + Xdc(1)*Yqz(h)+Xqz(h)*Ydc(1); 
%         else
%             %%%%%%%%%%%%%%%%% POSITIVE (Ydc*Xp) %%%%%%%%%%%%%%%%%%%
%             if(Xmp ~= 0)
%                 V_ABC = [Ydc(1)*Xmp*(cos(Xap)       +1i*sin(Xap));
%                          Ydc(2)*Xmp*(cos(Xap-2*pi/3)+1i*sin(Xap-2*pi/3));
%                          Ydc(3)*Xmp*(cos(Xap+2*pi/3)+1i*sin(Xap+2*pi/3))];
%                 V_012 = T*V_ABC/3;
% 
%                 Zdz(h) = Zdz(h) + real(V_012(1)); Zqz(h) = Zqz(h) + imag(V_012(1));
%                 Zdp(h) = Zdp(h) + real(V_012(2)); Zqp(h) = Zqp(h) + imag(V_012(2));
%                 Zdn(h) = Zdn(h) - real(V_012(3)); Zqn(h) = Zqn(h) + imag(V_012(3));
%             end
%             %%%%%%%%%%%%%%%%% POSITIVE (Xdc*Yp) %%%%%%%%%%%%%%%%%%%
%             if(Ymp ~= 0)
%             V_ABC = [Xdc(1)*Ymp*(cos(Yap)       +1i*sin(Yap));
%                      Xdc(2)*Ymp*(cos(Yap-2*pi/3)+1i*sin(Yap-2*pi/3));
%                      Xdc(3)*Ymp*(cos(Yap+2*pi/3)+1i*sin(Yap+2*pi/3))];
%             V_012 = T*V_ABC/3;
% 
%             Zdz(h) = Zdz(h) + real(V_012(1)); Zqz(h) = Zqz(h) + imag(V_012(1));
%             Zdp(h) = Zdp(h) + real(V_012(2)); Zqp(h) = Zqp(h) + imag(V_012(2));
%             Zdn(h) = Zdn(h) - real(V_012(3)); Zqn(h) = Zqn(h) + imag(V_012(3));
%             end
%             %%%%%%%%%%%%%%%%% NEGATIVE (Ydc*Xn) %%%%%%%%%%%%%%%%%%%
%             if(Xmn ~= 0)
%                 V_ABC = [Ydc(1)*Xmn*(cos(Xan)       +1i*sin(Xan));
%                          Ydc(2)*Xmn*(cos(Xan+2*pi/3)+1i*sin(Xan+2*pi/3));
%                          Ydc(3)*Xmn*(cos(Xan-2*pi/3)+1i*sin(Xan-2*pi/3))];
%                 V_012 = T*V_ABC/3;
% 
%                 Zdz(h) = Zdz(h) + real(V_012(1)); Zqz(h) = Zqz(h) + imag(V_012(1));
%                 Zdp(h) = Zdp(h) + real(V_012(2)); Zqp(h) = Zqp(h) + imag(V_012(2));
%                 Zdn(h) = Zdn(h) - real(V_012(3)); Zqn(h) = Zqn(h) + imag(V_012(3));
%             end
%             %%%%%%%%%%%%%%%%% NEGATIVE (Xdc*Yn) %%%%%%%%%%%%%%%%%%%
%             if(Ymn ~= 0)
%             V_ABC = [Xdc(1)*Ymn*(cos(Yan)       +1i*sin(Yan));
%                      Xdc(2)*Ymn*(cos(Yan+2*pi/3)+1i*sin(Yan+2*pi/3));
%                      Xdc(3)*Ymn*(cos(Yan-2*pi/3)+1i*sin(Yan-2*pi/3))];
%             V_012 = T*V_ABC/3;
% 
%             Zdz(h) = Zdz(h) + real(V_012(1)); Zqz(h) = Zqz(h) + imag(V_012(1));
%             Zdp(h) = Zdp(h) + real(V_012(2)); Zqp(h) = Zqp(h) + imag(V_012(2));
%             Zdn(h) = Zdn(h) - real(V_012(3)); Zqn(h) = Zqn(h) + imag(V_012(3));
%             end
%             %%%%%%%%%%%%%%%%%%%%%%%%%%%%%%%%%%%%%%%%%%%%%%%%%%%%%%
%             if(Xmz ~= 0)
%                 V_ABC = [Ydc(1)*Xmz*(cos(Xaz)+1i*sin(Xaz));
%                          Ydc(2)*Xmz*(cos(Xaz)+1i*sin(Xaz));
%                          Ydc(3)*Xmz*(cos(Xaz)+1i*sin(Xaz))];
%                 V_012 = T*V_ABC/3;
% 
%                 Zdz(h) = Zdz(h) + real(V_012(1)); Zqz(h) = Zqz(h) + imag(V_012(1));
%                 Zdp(h) = Zdp(h) + real(V_012(2)); Zqp(h) = Zqp(h) + imag(V_012(2));
%                 Zdn(h) = Zdn(h) - real(V_012(3)); Zqn(h) = Zqn(h) + imag(V_012(3));
%             end
%             %%%%%%%%%%%%%%%%%%%%%%%%%%%%%%%%%%%%%%%%%%%%%%%%%%%%%%
% 
%             if(Ymz ~= 0)
%                 V_ABC = [Xdc(1)*Ymz*(cos(Yaz)+1i*sin(Yaz));
%                          Xdc(2)*Ymz*(cos(Yaz)+1i*sin(Yaz));
%                          Xdc(3)*Ymz*(cos(Yaz)+1i*sin(Yaz))];
%                 V_012 = T*V_ABC/3;
%                 Zdz(h) = Zdz(h) + real(V_012(1)); Zqz(h) = Zqz(h) + imag(V_012(1));
%                 Zdp(h) = Zdp(h) + real(V_012(2)); Zqp(h) = Zqp(h) + imag(V_012(2));
%                 Zdn(h) = Zdn(h) - real(V_012(3)); Zqn(h) = Zqn(h) + imag(V_012(3));
%             end
%         end
%     end
% %     
% %     
% %    
% %     for h = 1 : 2*N
% %         if(h<=N)
% % 
% % %%%%%%%%%%%%%%%%%%%%%% h<=N ODD %%%%%%%%%%%%%%%%%%%%%%%%%%%%%%%%%%%%%%%%%
% %             if(mod(h,2)==1) 
% %                 %%%%%%%%%%%%%%%%% D3p (3ph+) %%%%%%%%%%%%%%%%%%%%%%%
% % 
% %                 %&%%%%%%%%%%%%%%%%%%%%%%%%%% PP + NN %%%%%%%%%%%%%%%%%%%%%%%%%%%
% %                 for i = 1 : h - 1
% %                    Zdp(h) = Zdp(h) - 0.5*(Xdn(i)*Yqn(h-i) + Xqn(i)*Ydn(h-i));                    
% %                    Zdn(h) = Zdn(h) - 0.5*(Xdp(i)*Yqp(h-i) + Xqp(i)*Ydp(h-i)); 
% %                    Zqp(h) = Zqp(h) - 0.5*(Xdn(i)*Ydn(h-i) - Xqn(i)*Yqn(h-i));                
% %                    Zqn(h) = Zqn(h) - 0.5*(Xdp(i)*Ydp(h-i) - Xqp(i)*Yqp(h-i)); 
% %                 end
% % 
% %                 for i = 1 : N - h
% %                     Zdz(h) = Zdz(h) + 0.5*(-Xdp(i)*Yqp(i+h) + Xqp(i)*Ydp(i+h) + Xdp(i+h)*Yqp(i) - Xqp(i+h)*Ydp(i) + Xdn(i)*Yqn(i+h) - Xqn(i)*Ydn(i+h) - Xdn(i+h)*Yqn(i) + Xqn(i+h)*Ydn(i));  
% %                     Zqz(h) = Zqz(h) + 0.5*(+Xdp(i)*Ydp(i+h) + Xqp(i)*Yqp(i+h) + Xdp(i+h)*Ydp(i) + Xqp(i+h)*Yqp(i) + Xdn(i)*Ydn(i+h) + Xqn(i)*Yqn(i+h) + Xdn(i+h)*Ydn(i) + Xqn(i+h)*Yqn(i));    
% %                 end
% %                 %&%%%%%%%%%%%%%%%%%%%%%%%%%% PP + NN %%%%%%%%%%%%%%%%%%%%%%%%%%%
% % 
% %                 for k = 1 : (N + mod(N+1,2) - h)/2
% %                     i = 2*k-1;
% %                     j = i+h;
% % 
% %                     Zdz(h)  = Zdz(h)  + 0.5*(-Xdz(i)*Yqz(j) + Xqz(i)*Ydz(j) + Xdz(j)*Yqz(i) - Xqz(j)*Ydz(i));
% %                     Zqz(h)  = Zqz(h)  + 0.5*(+Xdz(i)*Ydz(j) + Xqz(i)*Yqz(j) + Xdz(j)*Ydz(i) + Xqz(j)*Yqz(i)); 
% % 
% %                     Zdp(h) = Zdp(h) + 0.5*(-Xdp(i)*Yqn(j) - Xqp(i)*Ydn(j) - Xdn(j)*Yqp(i) - Xqn(j)*Ydp(i)); 
% %                     Zdp(h) = Zdp(h) + 0.5*(-Xdz(i)*Yqp(j) + Xqz(i)*Ydp(j) + Xdp(j)*Yqz(i) - Xqp(j)*Ydz(i));    
% %                     Zdp(h) = Zdp(h) + 0.5*(+Xdn(i)*Yqz(j) + Xqn(i)*Ydz(j) + Xdz(j)*Yqn(i) + Xqz(j)*Ydn(i));
% %                     
% %                     Zqp(h) = Zqp(h) + 0.5*(-Xdp(i)*Ydn(j) + Xqp(i)*Yqn(j) - Xdn(j)*Ydp(i) + Xqn(j)*Yqp(i));  
% %                     Zqp(h) = Zqp(h) + 0.5*(+Xdz(i)*Ydp(j) + Xqz(i)*Yqp(j) + Xdp(j)*Ydz(i) + Xqp(j)*Yqz(i));     
% %                     Zqp(h) = Zqp(h) + 0.5*(-Xdn(i)*Ydz(j) + Xqn(i)*Yqz(j) - Xdz(j)*Ydn(i) + Xqz(j)*Yqn(i));
% % 
% %                     Zdn(h) = Zdn(h) + 0.5*(+Xdp(i)*Yqz(j) - Xqp(i)*Ydz(j) - Xdz(j)*Yqp(i) + Xqz(j)*Ydp(i));             
% %                     Zdn(h) = Zdn(h) + 0.5*(+Xdz(i)*Yqn(j) + Xqz(i)*Ydn(j) + Xdn(j)*Yqz(i) + Xqn(j)*Ydz(i));
% %                     Zdn(h) = Zdn(h) + 0.5*(-Xdn(i)*Yqp(j) - Xqn(i)*Ydp(j) - Xdp(j)*Yqn(i) - Xqp(j)*Ydn(i)); 
% % 
% %                     Zqn(h) = Zqn(h) + 0.5*(+Xdp(i)*Ydz(j) + Xqp(i)*Yqz(j) + Xdz(j)*Ydp(i) + Xqz(j)*Yqp(i)); 
% %                     Zqn(h) = Zqn(h) + 0.5*(-Xdz(i)*Ydn(j) + Xqz(i)*Yqn(j) - Xdn(j)*Ydz(i) + Xqn(j)*Yqz(i)); 
% %                     Zqn(h) = Zqn(h) + 0.5*(-Xdn(i)*Ydp(j) + Xqn(i)*Yqp(j) - Xdp(j)*Ydn(i) + Xqp(j)*Yqn(i));  
% %                 end
% % 
% %                 for k = 1 : (N + mod(N,2) - h - 1)/2
% %                     i = 2*k;
% %                     j = i+h;
% %                     
% %                     Zdz(h) = Zdz(h)   + 0.5*(-Xdz(i)*Yqz(j) + Xqz(i)*Ydz(j) + Xdz(j)*Yqz(i) - Xqz(j)*Ydz(i));
% %                     Zqz(h) = Zqz(h)   + 0.5*(+Xdz(i)*Ydz(j) + Xqz(i)*Yqz(j) + Xdz(j)*Ydz(i) + Xqz(j)*Yqz(i)); 
% % 
% %                     Zdp(h) = Zdp(h) + 0.5*(-Xdp(i)*Yqn(j) - Xqp(i)*Ydn(j) - Xdn(j)*Yqp(i) - Xqn(j)*Ydp(i)); 
% %                     Zqp(h) = Zqp(h) + 0.5*(-Xdp(i)*Ydn(j) + Xqp(i)*Yqn(j) - Xdn(j)*Ydp(i) + Xqn(j)*Yqp(i));  
% %                     Zdn(h) = Zdn(h) + 0.5*(-Xdn(i)*Yqp(j) - Xqn(i)*Ydp(j) - Xdp(j)*Yqn(i) - Xqp(j)*Ydn(i)); 
% %                     Zqn(h) = Zqn(h) + 0.5*(-Xdn(i)*Ydp(j) + Xqn(i)*Yqp(j) - Xdp(j)*Ydn(i) + Xqp(j)*Yqn(i));                                          
% % 
% %                     Zdp(h) = Zdp(h) + 0.5*(-Xdz(i)*Yqp(j) + Xqz(i)*Ydp(j) + Xdp(j)*Yqz(i) - Xqp(j)*Ydz(i));
% %                     Zqp(h) = Zqp(h) + 0.5*(+Xdz(i)*Ydp(j) + Xqz(i)*Yqp(j) + Xdp(j)*Ydz(i) + Xqp(j)*Yqz(i));                     
% %                     Zdn(h) = Zdn(h) + 0.5*(+Xdp(i)*Yqz(j) - Xqp(i)*Ydz(j) - Xdz(j)*Yqp(i) + Xqz(j)*Ydp(i));
% %                     Zqn(h) = Zqn(h) + 0.5*(+Xdp(i)*Ydz(j) + Xqp(i)*Yqz(j) + Xdz(j)*Ydp(i) + Xqz(j)*Yqp(i));   
% % 
% %                     Zdp(h) = Zdp(h) + 0.5*(+Xdn(i)*Yqz(j) + Xqn(i)*Ydz(j) + Xdz(j)*Yqn(i) + Xqz(j)*Ydn(i));
% %                     Zqp(h) = Zqp(h) + 0.5*(-Xdn(i)*Ydz(j) + Xqn(i)*Yqz(j) - Xdz(j)*Ydn(i) + Xqz(j)*Yqn(i));                
% %                     Zdn(h) = Zdn(h) + 0.5*(+Xdz(i)*Yqn(j) + Xqz(i)*Ydn(j) + Xdn(j)*Yqz(i) + Xqn(j)*Ydz(i));
% %                     Zqn(h) = Zqn(h) + 0.5*(-Xdz(i)*Ydn(j) + Xqz(i)*Yqn(j) - Xdn(j)*Ydz(i) + Xqn(j)*Yqz(i)); 
% % 
% %                 end
% % 
% %                 for k = (h-1)/2:-1:1
% %                     i = k;
% %                     j = h-i;  
% %                     
% %                     Zdz(h) = Zdz(h) + 0.5*(+Xdp(i)*Yqn(j)-Xqp(i)*Ydn(j)-Xdn(j)*Yqp(i)+Xqn(j)*Ydp(i));
% %                     Zqz(h) = Zqz(h) + 0.5*(+Xdp(i)*Ydn(j)+Xqp(i)*Yqn(j)+Xdn(j)*Ydp(i)+Xqn(j)*Yqp(i));
% %                     Zdz(h) = Zdz(h) + 0.5*(+Xdp(j)*Yqn(i)-Xqp(j)*Ydn(i)-Xdn(i)*Yqp(j)+Xqn(i)*Ydp(j));
% %                     Zqz(h) = Zqz(h) + 0.5*(+Xdp(j)*Ydn(i)+Xqp(j)*Yqn(i)+Xdn(i)*Ydp(j)+Xqn(i)*Yqp(j)); 
% %                     Zdz(h) = Zdz(h) + 0.5*(+Xdz(i)*Yqz(j)+Xqz(i)*Ydz(j)+Xdz(j)*Yqz(i)+Xqz(j)*Ydz(i));
% %                     Zqz(h) = Zqz(h) + 0.5*(-Xdz(i)*Ydz(j)+Xqz(i)*Yqz(j)-Xdz(j)*Ydz(i)+Xqz(j)*Yqz(i));    
% %                         
% %                         
% %                     Zdp(h) = Zdp(h) + 0.5*(+Xdz(i)*Yqp(j)+Xqz(i)*Ydp(j)+Xdz(j)*Yqp(i)+Xqz(j)*Ydp(i));
% %                     Zqp(h) = Zqp(h) + 0.5*(-Xdz(i)*Ydp(j)+Xqz(i)*Yqp(j)-Xdz(j)*Ydp(i)+Xqz(j)*Yqp(i));
% %                     Zdp(h) = Zdp(h) + 0.5*(+Xdp(i)*Yqz(j)+Xqp(i)*Ydz(j)+Xdp(j)*Yqz(i)+Xqp(j)*Ydz(i));
% %                     Zqp(h) = Zqp(h) + 0.5*(-Xdp(i)*Ydz(j)+Xqp(i)*Yqz(j)-Xdp(j)*Ydz(i)+Xqp(j)*Yqz(i)); 
% %                     
% %                               
% %                     Zdn(h) = Zdn(h) + 0.5*(+Xdn(i)*Yqz(j)-Xqn(i)*Ydz(j)+Xdn(j)*Yqz(i)-Xqn(j)*Ydz(i));
% %                     Zqn(h) = Zqn(h) + 0.5*(+Xdn(i)*Ydz(j)+Xqn(i)*Yqz(j)+Xdn(j)*Ydz(i)+Xqn(j)*Yqz(i)); 
% %                     Zdn(h) = Zdn(h) + 0.5*(-Xdz(i)*Yqn(j)+Xqz(i)*Ydn(j)-Xdz(j)*Yqn(i)+Xqz(j)*Ydn(i));
% %                     Zqn(h) = Zqn(h) + 0.5*(+Xdz(i)*Ydn(j)+Xqz(i)*Yqn(j)+Xdz(j)*Ydn(i)+Xqz(j)*Yqn(i)); 
% %                 end
% % %%%%%%%%%%%%%%%%%%%%%% h<=N EVEN %%%%%%%%%%%%%%%%%%%%%%%%%%%%%%%%%%%%%%%%%           
% %             else 
% %                
% %                 Zdp(h) = Zdp(h) + 0.5*(-Xdn(h/2)*Yqn(h/2)-Xqn(h/2)*Ydn(h/2));   
% %                 Zqp(h) = Zqp(h) + 0.5*(-Xdn(h/2)*Ydn(h/2)+Xqn(h/2)*Yqn(h/2)); 
% %                 Zdn(h) = Zdn(h) + 0.5*(-Xdp(h/2)*Yqp(h/2)-Xqp(h/2)*Ydp(h/2));   
% %                 Zqn(h) = Zqn(h) + 0.5*(-Xdp(h/2)*Ydp(h/2)+Xqp(h/2)*Yqp(h/2));   
% % 
% %                 Zdz(h)  = Zdz(h)  + 0.5*(+Xdz(h/2)*Yqz(h/2)+Xqz(h/2)*Ydz(h/2));
% %                 Zqz(h)  = Zqz(h)  + 0.5*(-Xdz(h/2)*Ydz(h/2)+Xqz(h/2)*Yqz(h/2));
% % 
% %                 Zdp(h) = Zdp(h) + 0.5*(+Xdz(h/2)*Yqp(h/2)+Xqz(h/2)*Ydp(h/2)+Xdp(h/2)*Yqz(h/2)+Xqp(h/2)*Ydz(h/2));   
% %                 Zqp(h) = Zqp(h) + 0.5*(-Xdz(h/2)*Ydp(h/2)+Xqz(h/2)*Yqp(h/2)-Xdp(h/2)*Ydz(h/2)+Xqp(h/2)*Yqz(h/2)); 
% %                 Zdn(h) = Zdn(h) + 0.5*(+Xdn(h/2)*Yqz(h/2)-Xqn(h/2)*Ydz(h/2)-Xdz(h/2)*Yqn(h/2)+Xqz(h/2)*Ydn(h/2));   
% %                 Zqn(h) = Zqn(h) + 0.5*(+Xdn(h/2)*Ydz(h/2)+Xqn(h/2)*Yqz(h/2)+Xdz(h/2)*Ydn(h/2)+Xqz(h/2)*Yqn(h/2));    
% %                 
% %                 for k = 1:N-h
% %                     i = k;
% %                     j = h+i;
% %                 
% %                     Zdz(h) = Zdz(h)   + 0.5*(+Xdp(j)*Yqp(i) - Xqp(j)*Ydp(i) - Xdp(i)*Yqp(j) + Xqp(i)*Ydp(j));
% %                     Zqz(h) = Zqz(h)   + 0.5*(+Xdp(j)*Ydp(i) + Xqp(j)*Yqp(i) + Xdp(i)*Ydp(j) + Xqp(i)*Yqp(j));                                           
% %                     Zdz(h) = Zdz(h)   + 0.5*(+Xdn(i)*Yqn(j) - Xqn(i)*Ydn(j) - Xdn(j)*Yqn(i) + Xqn(j)*Ydn(i));
% %                     Zqz(h) = Zqz(h)   + 0.5*(+Xdn(i)*Ydn(j) + Xqn(i)*Yqn(j) + Xdn(j)*Ydn(i) + Xqn(j)*Yqn(i));  
% %                     Zdz(h) = Zdz(h)   + 0.5*(-Xdz(i)*Yqz(j) + Xqz(i)*Ydz(j) + Xdz(j)*Yqz(i) - Xqz(j)*Ydz(i));
% %                     Zqz(h) = Zqz(h)   + 0.5*(+Xdz(i)*Ydz(j) + Xqz(i)*Yqz(j) + Xdz(j)*Ydz(i) + Xqz(j)*Yqz(i)); 
% %                                        
% %                     Zdp(h) = Zdp(h) + 0.5*(-Xdp(i)*Yqn(j) - Xqp(i)*Ydn(j) - Xdn(j)*Yqp(i) - Xqn(j)*Ydp(i)); 
% %                     Zqp(h) = Zqp(h) + 0.5*(-Xdp(i)*Ydn(j) + Xqp(i)*Yqn(j) - Xdn(j)*Ydp(i) + Xqn(j)*Yqp(i)); 
% %                     Zdn(h) = Zdn(h) + 0.5*(-Xdn(i)*Yqp(j) - Xqn(i)*Ydp(j) - Xdp(j)*Yqn(i) - Xqp(j)*Ydn(i)); 
% %                     Zqn(h) = Zqn(h) + 0.5*(-Xdn(i)*Ydp(j) + Xqn(i)*Yqp(j) - Xdp(j)*Ydn(i) + Xqp(j)*Yqn(i)); 
% %                         
% %                     Zdp(h) = Zdp(h) + 0.5*(+Xdp(j)*Yqz(i) - Xqp(j)*Ydz(i) - Xdz(i)*Yqp(j) + Xqz(i)*Ydp(j));
% %                     Zqp(h) = Zqp(h) + 0.5*(+Xdp(j)*Ydz(i) + Xqp(j)*Yqz(i) + Xdz(i)*Ydp(j) + Xqz(i)*Yqp(j)); 
% %                     Zdn(h) = Zdn(h) + 0.5*(+Xdp(i)*Yqz(j) - Xqp(i)*Ydz(j) - Xdz(j)*Yqp(i) + Xqz(j)*Ydp(i));
% %                     Zqn(h) = Zqn(h) + 0.5*(+Xdp(i)*Ydz(j) + Xqp(i)*Yqz(j) + Xdz(j)*Ydp(i) + Xqz(j)*Yqp(i)); 
% %                     
% %                     Zdp(h) = Zdp(h) + 0.5*(+Xdn(i)*Yqz(j) + Xqn(i)*Ydz(j) + Xdz(j)*Yqn(i) + Xqz(j)*Ydn(i));
% %                     Zqp(h) = Zqp(h) + 0.5*(-Xdn(i)*Ydz(j) + Xqn(i)*Yqz(j) - Xdz(j)*Ydn(i) + Xqz(j)*Yqn(i)); 
% %                     Zdn(h) = Zdn(h) + 0.5*(+Xdn(j)*Yqz(i) + Xqn(j)*Ydz(i) + Xdz(i)*Yqn(j) + Xqz(i)*Ydn(j));
% %                     Zqn(h) = Zqn(h) + 0.5*(-Xdn(j)*Ydz(i) + Xqn(j)*Yqz(i) - Xdz(i)*Ydn(j) + Xqz(i)*Yqn(j)); 
% %                 end
% % 
% %                 for k = h/2-1:-1:1
% %                     i = k;
% %                     j = h-i;   
% % 
% %                     Zdz(h) = Zdz(h)   + 0.5*(+Xdp(i)*Yqn(j) - Xqp(i)*Ydn(j) + Xdp(j)*Yqn(i) - Xqp(j)*Ydn(i));
% %                     Zdz(h) = Zdz(h)   + 0.5*(-Xdn(i)*Yqp(j) + Xqn(i)*Ydp(j) - Xdn(j)*Yqp(i) + Xqn(j)*Ydp(i));      
% %                     Zdz(h) = Zdz(h)   + 0.5*(+Xdz(i)*Yqz(j) + Xqz(i)*Ydz(j) + Xdz(j)*Yqz(i) + Xqz(j)*Ydz(i));
% %                     
% %                     Zqz(h) = Zqz(h)   + 0.5*(+Xdp(i)*Ydn(j) + Xqp(i)*Yqn(j) + Xdp(j)*Ydn(i) + Xqp(j)*Yqn(i)); 
% %                     Zqz(h) = Zqz(h)   + 0.5*(+Xdn(i)*Ydp(j) + Xqn(i)*Yqp(j) + Xdn(j)*Ydp(i) + Xqn(j)*Yqp(i));
% %                     Zqz(h) = Zqz(h)   + 0.5*(-Xdz(i)*Ydz(j) + Xqz(i)*Yqz(j) - Xdz(j)*Ydz(i) + Xqz(j)*Yqz(i)); 
% %                     
% %                     Zdp(h) = Zdp(h) + 0.5*(+Xdp(i)*Yqz(j) + Xqp(i)*Ydz(j) + Xdp(j)*Yqz(i) + Xqp(j)*Ydz(i)); 
% %                     Zdp(h) = Zdp(h) + 0.5*(-Xdn(i)*Yqn(j) - Xqn(i)*Ydn(j) - Xdn(j)*Yqn(i) - Xqn(j)*Ydn(i)); 
% %                     Zdp(h) = Zdp(h) + 0.5*(+Xdz(i)*Yqp(j) + Xqz(i)*Ydp(j) + Xdz(j)*Yqp(i) + Xqz(j)*Ydp(i));
% %                     
% %                     Zqp(h) = Zqp(h) + 0.5*(-Xdp(i)*Ydz(j) + Xqp(i)*Yqz(j) - Xdp(j)*Ydz(i) + Xqp(j)*Yqz(i)); 
% %                     Zqp(h) = Zqp(h) + 0.5*(-Xdn(i)*Ydn(j) + Xqn(i)*Yqn(j) - Xdn(j)*Ydn(i) + Xqn(j)*Yqn(i));
% %                     Zqp(h) = Zqp(h) + 0.5*(-Xdz(i)*Ydp(j) + Xqz(i)*Yqp(j) - Xdz(j)*Ydp(i) + Xqz(j)*Yqp(i));  
% %                     
% %                     Zdn(h) = Zdn(h) + 0.5*(-Xdp(i)*Yqp(j) - Xqp(i)*Ydp(j) - Xdp(j)*Yqp(i) - Xqp(j)*Ydp(i));
% %                     Zdn(h) = Zdn(h) + 0.5*(+Xdn(i)*Yqz(j) - Xqn(i)*Ydz(j) + Xdn(j)*Yqz(i) - Xqn(j)*Ydz(i));
% %                     Zdn(h) = Zdn(h) + 0.5*(-Xdz(i)*Yqn(j) + Xqz(i)*Ydn(j) - Xdz(j)*Yqn(i) + Xqz(j)*Ydn(i));
% %                     
% %                     Zqn(h) = Zqn(h) + 0.5*(-Xdp(i)*Ydp(j) + Xqp(i)*Yqp(j) - Xdp(j)*Ydp(i) + Xqp(j)*Yqp(i));  
% %                     Zqn(h) = Zqn(h) + 0.5*(+Xdn(i)*Ydz(j) + Xqn(i)*Yqz(j) + Xdn(j)*Ydz(i) + Xqn(j)*Yqz(i));
% %                     Zqn(h) = Zqn(h) + 0.5*(+Xdz(i)*Ydn(j) + Xqz(i)*Yqn(j) + Xdz(j)*Ydn(i) + Xqz(j)*Yqn(i)); 
% %                 end
% %             end
% % %%%%%%%%%%%%%%%%%%%%%%%%%%%% h>N  %%%%%%%%%%%%%%%%%%%%%%%%%%%%%%%%%%%%%%%%% 
% %         else %h>N
% %             
% %             
% %             %%%%%%%%%%%%%%%%%%%%%%%%%%% PP + NN %%%%%%%%%%%%%%%%%%%%%%%%%%%
% %             for i = h-N : N
% %                 Zdp(h) = Zdp(h) - 0.5*(Xdn(i)*Yqn(h-i) + Xqn(i)*Ydn(h-i));                
% %                 Zdn(h) = Zdn(h) - 0.5*(Xdp(i)*Yqp(h-i) + Xqp(i)*Ydp(h-i));                     
% %                 Zqp(h) = Zqp(h) - 0.5*(Xdn(i)*Ydn(h-i) - Xqn(i)*Yqn(h-i));                      
% %                 Zqn(h) = Zqn(h) - 0.5*(Xdp(i)*Ydp(h-i) - Xqp(i)*Yqp(h-i));   
% %             end
% %             %%%%%%%%%%%%%%%%%%%%%%%%%%% PP + NN %%%%%%%%%%%%%%%%%%%%%%%%%%%
% % 
% %             if(mod(h,2)==1) %%%%%%%%%%% h>N ODD %%%%%%%%%%%%%%%%%%%
% % 
% %                 for k = (h-1)/2:-1:h-N
% %                     i = k;
% %                     j = h-i;
% %                     
% %                     Zdz(h) = Zdz(h) + 0.5*(+Xdp(i)*Yqn(j)-Xqp(i)*Ydn(j)-Xdn(j)*Yqp(i)+Xqn(j)*Ydp(i));                  
% %                     Zdz(h) = Zdz(h) + 0.5*(+Xdp(j)*Yqn(i)-Xqp(j)*Ydn(i)-Xdn(i)*Yqp(j)+Xqn(i)*Ydp(j));
% %                     Zdz(h) = Zdz(h) + 0.5*(+Xdz(i)*Yqz(j)+Xqz(i)*Ydz(j)+Xdz(j)*Yqz(i)+Xqz(j)*Ydz(i));
% %                     
% %                     Zqz(h) = Zqz(h) + 0.5*(-Xdz(i)*Ydz(j)+Xqz(i)*Yqz(j)-Xdz(j)*Ydz(i)+Xqz(j)*Yqz(i));
% %                     Zqz(h) = Zqz(h) + 0.5*(+Xdp(i)*Ydn(j)+Xqp(i)*Yqn(j)+Xdn(j)*Ydp(i)+Xqn(j)*Yqp(i));
% %                     Zqz(h) = Zqz(h) + 0.5*(+Xdp(j)*Ydn(i)+Xqp(j)*Yqn(i)+Xdn(i)*Ydp(j)+Xqn(i)*Yqp(j));  
% %                     
% %                     Zdp(h) = Zdp(h) + 0.5*(+Xdp(i)*Yqz(j)+Xqp(i)*Ydz(j)+Xdp(j)*Yqz(i)+Xqp(j)*Ydz(i));
% %                     Zdp(h) = Zdp(h) + 0.5*(+Xdz(i)*Yqp(j)+Xqz(i)*Ydp(j)+Xdz(j)*Yqp(i)+Xqz(j)*Ydp(i));
% %                     
% %                     Zqp(h) = Zqp(h) + 0.5*(-Xdp(i)*Ydz(j)+Xqp(i)*Yqz(j)-Xdp(j)*Ydz(i)+Xqp(j)*Yqz(i)); 
% %                     Zqp(h) = Zqp(h) + 0.5*(-Xdz(i)*Ydp(j)+Xqz(i)*Yqp(j)-Xdz(j)*Ydp(i)+Xqz(j)*Yqp(i));     
% %                                        
% %                     Zdn(h) = Zdn(h) + 0.5*(+Xdn(i)*Yqz(j)-Xqn(i)*Ydz(j)+Xdn(j)*Yqz(i)-Xqn(j)*Ydz(i));
% %                     Zdn(h) = Zdn(h) + 0.5*(-Xdz(i)*Yqn(j)+Xqz(i)*Ydn(j)-Xdz(j)*Yqn(i)+Xqz(j)*Ydn(i));
% %                     
% %                     Zqn(h) = Zqn(h) + 0.5*(+Xdn(i)*Ydz(j)+Xqn(i)*Yqz(j)+Xdn(j)*Ydz(i)+Xqn(j)*Yqz(i));
% %                     Zqn(h) = Zqn(h) + 0.5*(+Xdz(i)*Ydn(j)+Xqz(i)*Yqn(j)+Xdz(j)*Ydn(i)+Xqz(j)*Yqn(i));    
% % 
% %                 end
% % 
% %             else %%%%%%%%%%% h>N EVEN %%%%%%%%%%%%%%%%%%%
% % 
% %                 Zdz(h)  = Zdz(h)  + 0.5*(+Xdz(h/2)*Yqz(h/2)+Xqz(h/2)*Ydz(h/2));
% %                 Zqz(h)  = Zqz(h)  + 0.5*(-Xdz(h/2)*Ydz(h/2)+Xqz(h/2)*Yqz(h/2));
% %                 
% %                 Zdp(h) = 0.5*(-Xdn(h/2)*Yqn(h/2)-Xqn(h/2)*Ydn(h/2));          
% %                 Zdp(h) = Zdp(h) + 0.5*(+Xdp(h/2)*Yqz(h/2)+Xqp(h/2)*Ydz(h/2));                
% %                 Zdp(h) = Zdp(h) + 0.5*(+Xdz(h/2)*Yqp(h/2)+Xqz(h/2)*Ydp(h/2));    
% %                 
% %                 Zqp(h) = 0.5*(-Xdn(h/2)*Ydn(h/2)+Xqn(h/2)*Yqn(h/2));             
% %                 Zqp(h) = Zqp(h) + 0.5*(-Xdp(h/2)*Ydz(h/2)+Xqp(h/2)*Yqz(h/2));        
% %                 Zqp(h) = Zqp(h) + 0.5*(-Xdz(h/2)*Ydp(h/2)+Xqz(h/2)*Yqp(h/2)); 
% %                 
% %                 Zdn(h) = 0.5*(-Xdp(h/2)*Yqp(h/2)-Xqp(h/2)*Ydp(h/2)); 
% %                 Zdn(h) = Zdn(h) + 0.5*(+Xdn(h/2)*Yqz(h/2)-Xqn(h/2)*Ydz(h/2));
% %                 Zdn(h) = Zdn(h) + 0.5*(-Xdz(h/2)*Yqn(h/2)+Xqz(h/2)*Ydn(h/2));
% %                                
% %                 Zqn(h) = 0.5*(-Xdp(h/2)*Ydp(h/2)+Xqp(h/2)*Yqp(h/2)); 
% %                 Zqn(h) = Zqn(h) + 0.5*(+Xdn(h/2)*Ydz(h/2)+Xqn(h/2)*Yqz(h/2));        
% %                 Zqn(h) = Zqn(h) + 0.5*(+Xdz(h/2)*Ydn(h/2)+Xqz(h/2)*Yqn(h/2)); 
% % 
% %                 for i = (h+2)/2:N
% %                     j = h-i;
% %                     Zdz(h)  = Zdz(h)  + 0.5*(+Xdp(i)*Yqn(j)-Xqp(i)*Ydn(j)+Xdp(j)*Yqn(i)-Xqp(j)*Ydn(i));
% %                     Zdz(h)  = Zdz(h)  + 0.5*(-Xdn(i)*Yqp(j)+Xqn(i)*Ydp(j)-Xdn(j)*Yqp(i)+Xqn(j)*Ydp(i));
% %                     Zdz(h)  = Zdz(h)  + 0.5*(+Xdz(i)*Yqz(j)+Xqz(i)*Ydz(j)+Xdz(j)*Yqz(i)+Xqz(j)*Ydz(i));
% %                     
% %                     Zqz(h)  = Zqz(h)  + 0.5*(+Xdp(i)*Ydn(j)+Xqp(i)*Yqn(j)+Xdp(j)*Ydn(i)+Xqp(j)*Yqn(i));                      
% %                     Zqz(h)  = Zqz(h)  + 0.5*(+Xdn(i)*Ydp(j)+Xqn(i)*Yqp(j)+Xdn(j)*Ydp(i)+Xqn(j)*Yqp(i));  
% %                     Zqz(h)  = Zqz(h)  + 0.5*(-Xdz(i)*Ydz(j)+Xqz(i)*Yqz(j)-Xdz(j)*Ydz(i)+Xqz(j)*Yqz(i));
% %                     
% %                     Zdp(h) = Zdp(h) + 0.5*(+Xdp(i)*Yqz(j)+Xqp(i)*Ydz(j)+Xdp(j)*Yqz(i)+Xqp(j)*Ydz(i));  
% %                     Zdp(h) = Zdp(h) + 0.5*(-Xdn(i)*Yqn(j)-Xqn(i)*Ydn(j)-Xdn(j)*Yqn(i)-Xqn(j)*Ydn(i));             
% %                     Zdp(h) = Zdp(h) + 0.5*(+Xdz(i)*Yqp(j)+Xqz(i)*Ydp(j)+Xdz(j)*Yqp(i)+Xqz(j)*Ydp(i));           
% %                     
% %                     Zqp(h) = Zqp(h) + 0.5*(-Xdp(i)*Ydz(j)+Xqp(i)*Yqz(j)-Xdp(j)*Ydz(i)+Xqp(j)*Yqz(i));
% %                     Zqp(h) = Zqp(h) + 0.5*(-Xdn(i)*Ydn(j)+Xqn(i)*Yqn(j)-Xdn(j)*Ydn(i)+Xqn(j)*Yqn(i));    
% %                     Zqp(h) = Zqp(h) + 0.5*(-Xdz(i)*Ydp(j)+Xqz(i)*Yqp(j)-Xdz(j)*Ydp(i)+Xqz(j)*Yqp(i));   
% %                     
% %                     Zdn(h) = Zdn(h) + 0.5*(-Xdp(i)*Yqp(j)-Xqp(i)*Ydp(j)-Xdp(j)*Yqp(i)-Xqp(j)*Ydp(i));
% %                     Zdn(h) = Zdn(h) + 0.5*(+Xdn(i)*Yqz(j)-Xqn(i)*Ydz(j)+Xdn(j)*Yqz(i)-Xqn(j)*Ydz(i));
% %                     Zdn(h) = Zdn(h) + 0.5*(-Xdz(i)*Yqn(j)+Xqz(i)*Ydn(j)-Xdz(j)*Yqn(i)+Xqz(j)*Ydn(i));              
% %                     
% %                     Zqn(h) = Zqn(h) + 0.5*(-Xdp(i)*Ydp(j)+Xqp(i)*Yqp(j)-Xdp(j)*Ydp(i)+Xqp(j)*Yqp(i));
% %                     Zqn(h) = Zqn(h) + 0.5*(+Xdn(i)*Ydz(j)+Xqn(i)*Yqz(j)+Xdn(j)*Ydz(i)+Xqn(j)*Yqz(i)); 
% %                     Zqn(h) = Zqn(h) + 0.5*(+Xdz(i)*Ydn(j)+Xqz(i)*Yqn(j)+Xdz(j)*Ydn(i)+Xqz(j)*Yqn(i));  
% %                 end
% %             end
% %         end  
% %     end
% end
%     

% function [Zdc,Zdp,Zdn,Zdz,Zqp,Zqn,Zqz]  = MultDQN(Xdc, Xdp, Xdn, Xdz, Xqp, Xqn, Xqz, Ydc, Ydp, Ydn, Ydz, Yqp, Yqn, Yqz, N)
% 
%     Zdc = zeros(1,3);
%     a = -0.5+0.866i;
%     a2 = -0.5-0.866i;
%     T = [1 1 1;1 a a2;1 a2 a];
% 
%     Xdp = [Xdp; zeros(N-numel(Xdp),1)];
%     Ydp = [Ydp; zeros(N-numel(Ydp),1)];
%     Xqp = [Xqp; zeros(N-numel(Xqp),1)];
%     Yqp = [Yqp; zeros(N-numel(Yqp),1)];
%       
%     Xdn = [Xdn; zeros(N-numel(Xdn),1)];
%     Ydn = [Ydn; zeros(N-numel(Ydn),1)];
%     Xqn = [Xqn; zeros(N-numel(Xqn),1)];
%     Yqn = [Yqn; zeros(N-numel(Yqn),1)];
%     
%     Xdz = [Xdz; zeros(N-numel(Xdz),1)];
%     Ydz = [Ydz; zeros(N-numel(Ydz),1)];
%     Xqz = [Xqz; zeros(N-numel(Xqz),1)];
%     Yqz = [Yqz; zeros(N-numel(Yqz),1)];
%        
%     Zdp = zeros(1,2*N);
%     Zdn = zeros(1,2*N);
%     Zqp = zeros(1,2*N);
%     Zqn = zeros(1,2*N);
%     Zdz = zeros(1,2*N);
%     Zqz = zeros(1,2*N);
%    
%     Zdc = Xdc.*Ydc;
%     
%     
%     for h = 1 : N 
%         Zdc = Zdc + 0.5*(Xdp(h)*Ydp(h)+Xqp(h)*Yqp(h));
%         Zdc = Zdc + 0.5*(Xdn(h)*Ydn(h)+Xqn(h)*Yqn(h));
%         Zdc = Zdc + 0.5*(Xdz(h)*Ydz(h)+Xqz(h)*Yqz(h));
% 
%         Xmp = sqrt(Xdp(h)^2+Xqp(h)^2);
%         Xap = atan2(Xqp(h),+Xdp(h));  
%         Ymp = sqrt(Ydp(h)^2+Yqp(h)^2);
%         Yap = atan2(Yqp(h),+Ydp(h));  
% 
%         Xmn = sqrt(Xdn(h)^2+Xqn(h)^2);
%         Xan = atan2(Xqn(h),-Xdn(h));  
%         Ymn = sqrt(Ydn(h)^2+Yqn(h)^2);
%         Yan = atan2(Yqn(h),-Ydn(h));  
% 
%         Xmz = sqrt(Xdz(h)^2+Xqz(h)^2);
%         Xaz = atan2(Xqz(h),+Xdz(h));  
%         Ymz = sqrt(Ydz(h)^2+Yqz(h)^2);
%         Yaz = atan2(Yqz(h),+Ydz(h));  
% 
%         Zdz(2*h) = Zdz(2*h) + 0.5*Xmp*Ymn*sin(Xap+Yan);
%         Zqz(2*h) = Zqz(2*h) - 0.5*Xmp*Ymn*cos(Xap+Yan);
% 
%         Zdz(2*h) = Zdz(2*h) + 0.5*Xmn*Ymp*sin(Xan+Yap);
%         Zqz(2*h) = Zqz(2*h) - 0.5*Xmn*Ymp*cos(Xan+Yap);
% 
%         Zdc = Zdc + 0.5*Xmp*Ymn*[cos(Xap-Yan) cos(Xap-Yan-4*pi/3) cos(Xap-Yan+4*pi/3)];
%         Zdc = Zdc + 0.5*Xmn*Ymp*[cos(Xan-Yap) cos(Xan-Yap+4*pi/3) cos(Xan-Yap-4*pi/3)];
%         Zdc = Zdc + 0.5*Xmz*Ymp*[cos(Xaz-Yap) cos(Xaz-Yap-4*pi/3) cos(Xaz-Yap+4*pi/3)];
%         Zdc = Zdc + 0.5*Xmp*Ymz*[cos(Xap-Yaz) cos(Xap-Yaz+4*pi/3) cos(Xap-Yaz-4*pi/3)];
%         Zdc = Zdc + 0.5*Xmn*Ymz*[cos(Xan-Yaz) cos(Xan-Yaz-4*pi/3) cos(Xan-Yaz+4*pi/3)];
%         Zdc = Zdc + 0.5*Xmz*Ymn*[cos(Xaz-Yan) cos(Xaz-Yan+4*pi/3) cos(Xaz-Yan-4*pi/3)];
% 
%         if(all(Xdc == Xdc(1)) && all(Ydc == Ydc(1)))
%             Zdp(h) = Zdp(h) + Xdc(1)*Ydp(h)+Xdp(h)*Ydc(1);     
%             Zqp(h) = Zqp(h) + Xdc(1)*Yqp(h)+Xqp(h)*Ydc(1);  
%             Zdn(h) = Zdn(h) + Xdc(1)*Ydn(h)+Xdn(h)*Ydc(1);
%             Zqn(h) = Zqn(h) + Xdc(1)*Yqn(h)+Xqn(h)*Ydc(1);
%             Zdz(h) = Zdz(h) + Xdc(1)*Ydz(h)+Xdz(h)*Ydc(1);     
%             Zqz(h) = Zqz(h) + Xdc(1)*Yqz(h)+Xqz(h)*Ydc(1); 
%         else
%             %%%%%%%%%%%%%%%%% POSITIVE (Ydc*Xp) %%%%%%%%%%%%%%%%%%%
%             if(Xmp ~= 0)
%                 V_ABC = [Ydc(1)*Xmp*(cos(Xap)       +1i*sin(Xap));
%                          Ydc(2)*Xmp*(cos(Xap-2*pi/3)+1i*sin(Xap-2*pi/3));
%                          Ydc(3)*Xmp*(cos(Xap+2*pi/3)+1i*sin(Xap+2*pi/3))];
%                 V_012 = T*V_ABC/3;
% 
%                 Zdz(h) = Zdz(h) + real(V_012(1)); Zqz(h) = Zqz(h) + imag(V_012(1));
%                 Zdp(h) = Zdp(h) + real(V_012(2)); Zqp(h) = Zqp(h) + imag(V_012(2));
%                 Zdn(h) = Zdn(h) - real(V_012(3)); Zqn(h) = Zqn(h) + imag(V_012(3));
%             end
%             %%%%%%%%%%%%%%%%% POSITIVE (Xdc*Yp) %%%%%%%%%%%%%%%%%%%
%             if(Ymp ~= 0)
%             V_ABC = [Xdc(1)*Ymp*(cos(Yap)       +1i*sin(Yap));
%                      Xdc(2)*Ymp*(cos(Yap-2*pi/3)+1i*sin(Yap-2*pi/3));
%                      Xdc(3)*Ymp*(cos(Yap+2*pi/3)+1i*sin(Yap+2*pi/3))];
%             V_012 = T*V_ABC/3;
% 
%             Zdz(h) = Zdz(h) + real(V_012(1)); Zqz(h) = Zqz(h) + imag(V_012(1));
%             Zdp(h) = Zdp(h) + real(V_012(2)); Zqp(h) = Zqp(h) + imag(V_012(2));
%             Zdn(h) = Zdn(h) - real(V_012(3)); Zqn(h) = Zqn(h) + imag(V_012(3));
%             end
%             %%%%%%%%%%%%%%%%% NEGATIVE (Ydc*Xn) %%%%%%%%%%%%%%%%%%%
%             if(Xmn ~= 0)
%                 V_ABC = [Ydc(1)*Xmn*(cos(Xan)       +1i*sin(Xan));
%                          Ydc(2)*Xmn*(cos(Xan+2*pi/3)+1i*sin(Xan+2*pi/3));
%                          Ydc(3)*Xmn*(cos(Xan-2*pi/3)+1i*sin(Xan-2*pi/3))];
%                 V_012 = T*V_ABC/3;
% 
%                 Zdz(h) = Zdz(h) + real(V_012(1)); Zqz(h) = Zqz(h) + imag(V_012(1));
%                 Zdp(h) = Zdp(h) + real(V_012(2)); Zqp(h) = Zqp(h) + imag(V_012(2));
%                 Zdn(h) = Zdn(h) - real(V_012(3)); Zqn(h) = Zqn(h) + imag(V_012(3));
%             end
%             %%%%%%%%%%%%%%%%% NEGATIVE (Xdc*Yn) %%%%%%%%%%%%%%%%%%%
%             if(Ymn ~= 0)
%             V_ABC = [Xdc(1)*Ymn*(cos(Yan)       +1i*sin(Yan));
%                      Xdc(2)*Ymn*(cos(Yan+2*pi/3)+1i*sin(Yan+2*pi/3));
%                      Xdc(3)*Ymn*(cos(Yan-2*pi/3)+1i*sin(Yan-2*pi/3))];
%             V_012 = T*V_ABC/3;
% 
%             Zdz(h) = Zdz(h) + real(V_012(1)); Zqz(h) = Zqz(h) + imag(V_012(1));
%             Zdp(h) = Zdp(h) + real(V_012(2)); Zqp(h) = Zqp(h) + imag(V_012(2));
%             Zdn(h) = Zdn(h) - real(V_012(3)); Zqn(h) = Zqn(h) + imag(V_012(3));
%             end
%             %%%%%%%%%%%%%%%%%%%%%%%%%%%%%%%%%%%%%%%%%%%%%%%%%%%%%%
%             if(Xmz ~= 0)
%                 V_ABC = [Ydc(1)*Xmz*(cos(Xaz)+1i*sin(Xaz));
%                          Ydc(2)*Xmz*(cos(Xaz)+1i*sin(Xaz));
%                          Ydc(3)*Xmz*(cos(Xaz)+1i*sin(Xaz))];
%                 V_012 = T*V_ABC/3;
% 
%                 Zdz(h) = Zdz(h) + real(V_012(1)); Zqz(h) = Zqz(h) + imag(V_012(1));
%                 Zdp(h) = Zdp(h) + real(V_012(2)); Zqp(h) = Zqp(h) + imag(V_012(2));
%                 Zdn(h) = Zdn(h) - real(V_012(3)); Zqn(h) = Zqn(h) + imag(V_012(3));
%             end
%             %%%%%%%%%%%%%%%%%%%%%%%%%%%%%%%%%%%%%%%%%%%%%%%%%%%%%%
% 
%             if(Ymz ~= 0)
%                 V_ABC = [Xdc(1)*Ymz*(cos(Yaz)+1i*sin(Yaz));
%                          Xdc(2)*Ymz*(cos(Yaz)+1i*sin(Yaz));
%                          Xdc(3)*Ymz*(cos(Yaz)+1i*sin(Yaz))];
%                 V_012 = T*V_ABC/3;
%                 Zdz(h) = Zdz(h) + real(V_012(1)); Zqz(h) = Zqz(h) + imag(V_012(1));
%                 Zdp(h) = Zdp(h) + real(V_012(2)); Zqp(h) = Zqp(h) + imag(V_012(2));
%                 Zdn(h) = Zdn(h) - real(V_012(3)); Zqn(h) = Zqn(h) + imag(V_012(3));
%             end
%         end
%     end
%     
%     
%    
%     for h = 1 : 2*N
%         if(h<=N)
% 
% %%%%%%%%%%%%%%%%%%%%%% h<=N ODD %%%%%%%%%%%%%%%%%%%%%%%%%%%%%%%%%%%%%%%%%
%             if(mod(h,2)==1) 
%                 %%%%%%%%%%%%%%%%% D3p (3ph+) %%%%%%%%%%%%%%%%%%%%%%%
% 
%                 %&%%%%%%%%%%%%%%%%%%%%%%%%%% PP + NN %%%%%%%%%%%%%%%%%%%%%%%%%%%
%                 for i = 1 : h - 1
%                    Zdp(h) = Zdp(h) - 0.5*(Xdn(i)*Yqn(h-i) + Xqn(i)*Ydn(h-i));                    
%                    Zdn(h) = Zdn(h) - 0.5*(Xdp(i)*Yqp(h-i) + Xqp(i)*Ydp(h-i)); 
%                    Zqp(h) = Zqp(h) - 0.5*(Xdn(i)*Ydn(h-i) - Xqn(i)*Yqn(h-i));                
%                    Zqn(h) = Zqn(h) - 0.5*(Xdp(i)*Ydp(h-i) - Xqp(i)*Yqp(h-i)); 
%                 end
% 
%                 for i = 1 : N - h
%                     Zdz(h) = Zdz(h) + 0.5*(-Xdp(i)*Yqp(i+h) + Xqp(i)*Ydp(i+h) + Xdp(i+h)*Yqp(i) - Xqp(i+h)*Ydp(i) + Xdn(i)*Yqn(i+h) - Xqn(i)*Ydn(i+h) - Xdn(i+h)*Yqn(i) + Xqn(i+h)*Ydn(i));  
%                     Zqz(h) = Zqz(h) + 0.5*(+Xdp(i)*Ydp(i+h) + Xqp(i)*Yqp(i+h) + Xdp(i+h)*Ydp(i) + Xqp(i+h)*Yqp(i) + Xdn(i)*Ydn(i+h) + Xqn(i)*Yqn(i+h) + Xdn(i+h)*Ydn(i) + Xqn(i+h)*Yqn(i));    
%                 end
%                 %&%%%%%%%%%%%%%%%%%%%%%%%%%% PP + NN %%%%%%%%%%%%%%%%%%%%%%%%%%%
% 
%                 for k = 1 : (N + mod(N+1,2) - h)/2
%                     i = 2*k-1;
%                     j = i+h;
% 
%                     Zdz(h)  = Zdz(h)  + 0.5*(-Xdz(i)*Yqz(j) + Xqz(i)*Ydz(j) + Xdz(j)*Yqz(i) - Xqz(j)*Ydz(i));
%                     Zqz(h)  = Zqz(h)  + 0.5*(+Xdz(i)*Ydz(j) + Xqz(i)*Yqz(j) + Xdz(j)*Ydz(i) + Xqz(j)*Yqz(i)); 
% 
%                     Zdp(h) = Zdp(h) + 0.5*(-Xdp(i)*Yqn(j) - Xqp(i)*Ydn(j) - Xdn(j)*Yqp(i) - Xqn(j)*Ydp(i)); 
%                     Zdp(h) = Zdp(h) + 0.5*(-Xdz(i)*Yqp(j) + Xqz(i)*Ydp(j) + Xdp(j)*Yqz(i) - Xqp(j)*Ydz(i));    
%                     Zdp(h) = Zdp(h) + 0.5*(+Xdn(i)*Yqz(j) + Xqn(i)*Ydz(j) + Xdz(j)*Yqn(i) + Xqz(j)*Ydn(i));
%                     
%                     Zqp(h) = Zqp(h) + 0.5*(-Xdp(i)*Ydn(j) + Xqp(i)*Yqn(j) - Xdn(j)*Ydp(i) + Xqn(j)*Yqp(i));  
%                     Zqp(h) = Zqp(h) + 0.5*(+Xdz(i)*Ydp(j) + Xqz(i)*Yqp(j) + Xdp(j)*Ydz(i) + Xqp(j)*Yqz(i));     
%                     Zqp(h) = Zqp(h) + 0.5*(-Xdn(i)*Ydz(j) + Xqn(i)*Yqz(j) - Xdz(j)*Ydn(i) + Xqz(j)*Yqn(i));
% 
%                     Zdn(h) = Zdn(h) + 0.5*(+Xdp(i)*Yqz(j) - Xqp(i)*Ydz(j) - Xdz(j)*Yqp(i) + Xqz(j)*Ydp(i));             
%                     Zdn(h) = Zdn(h) + 0.5*(+Xdz(i)*Yqn(j) + Xqz(i)*Ydn(j) + Xdn(j)*Yqz(i) + Xqn(j)*Ydz(i));
%                     Zdn(h) = Zdn(h) + 0.5*(-Xdn(i)*Yqp(j) - Xqn(i)*Ydp(j) - Xdp(j)*Yqn(i) - Xqp(j)*Ydn(i)); 
% 
%                     Zqn(h) = Zqn(h) + 0.5*(+Xdp(i)*Ydz(j) + Xqp(i)*Yqz(j) + Xdz(j)*Ydp(i) + Xqz(j)*Yqp(i)); 
%                     Zqn(h) = Zqn(h) + 0.5*(-Xdz(i)*Ydn(j) + Xqz(i)*Yqn(j) - Xdn(j)*Ydz(i) + Xqn(j)*Yqz(i)); 
%                     Zqn(h) = Zqn(h) + 0.5*(-Xdn(i)*Ydp(j) + Xqn(i)*Yqp(j) - Xdp(j)*Ydn(i) + Xqp(j)*Yqn(i));  
%                 end
% 
%                 for k = 1 : (N + mod(N,2) - h - 1)/2
%                     i = 2*k;
%                     j = i+h;
%                     
%                     Zdz(h) = Zdz(h)   + 0.5*(-Xdz(i)*Yqz(j) + Xqz(i)*Ydz(j) + Xdz(j)*Yqz(i) - Xqz(j)*Ydz(i));
%                     Zqz(h) = Zqz(h)   + 0.5*(+Xdz(i)*Ydz(j) + Xqz(i)*Yqz(j) + Xdz(j)*Ydz(i) + Xqz(j)*Yqz(i)); 
% 
%                     Zdp(h) = Zdp(h) + 0.5*(-Xdp(i)*Yqn(j) - Xqp(i)*Ydn(j) - Xdn(j)*Yqp(i) - Xqn(j)*Ydp(i)); 
%                     Zqp(h) = Zqp(h) + 0.5*(-Xdp(i)*Ydn(j) + Xqp(i)*Yqn(j) - Xdn(j)*Ydp(i) + Xqn(j)*Yqp(i));  
%                     Zdn(h) = Zdn(h) + 0.5*(-Xdn(i)*Yqp(j) - Xqn(i)*Ydp(j) - Xdp(j)*Yqn(i) - Xqp(j)*Ydn(i)); 
%                     Zqn(h) = Zqn(h) + 0.5*(-Xdn(i)*Ydp(j) + Xqn(i)*Yqp(j) - Xdp(j)*Ydn(i) + Xqp(j)*Yqn(i));                                          
% 
%                     Zdp(h) = Zdp(h) + 0.5*(-Xdz(i)*Yqp(j) + Xqz(i)*Ydp(j) + Xdp(j)*Yqz(i) - Xqp(j)*Ydz(i));
%                     Zqp(h) = Zqp(h) + 0.5*(+Xdz(i)*Ydp(j) + Xqz(i)*Yqp(j) + Xdp(j)*Ydz(i) + Xqp(j)*Yqz(i));                     
%                     Zdn(h) = Zdn(h) + 0.5*(+Xdp(i)*Yqz(j) - Xqp(i)*Ydz(j) - Xdz(j)*Yqp(i) + Xqz(j)*Ydp(i));
%                     Zqn(h) = Zqn(h) + 0.5*(+Xdp(i)*Ydz(j) + Xqp(i)*Yqz(j) + Xdz(j)*Ydp(i) + Xqz(j)*Yqp(i));   
% 
%                     Zdp(h) = Zdp(h) + 0.5*(+Xdn(i)*Yqz(j) + Xqn(i)*Ydz(j) + Xdz(j)*Yqn(i) + Xqz(j)*Ydn(i));
%                     Zqp(h) = Zqp(h) + 0.5*(-Xdn(i)*Ydz(j) + Xqn(i)*Yqz(j) - Xdz(j)*Ydn(i) + Xqz(j)*Yqn(i));                
%                     Zdn(h) = Zdn(h) + 0.5*(+Xdz(i)*Yqn(j) + Xqz(i)*Ydn(j) + Xdn(j)*Yqz(i) + Xqn(j)*Ydz(i));
%                     Zqn(h) = Zqn(h) + 0.5*(-Xdz(i)*Ydn(j) + Xqz(i)*Yqn(j) - Xdn(j)*Ydz(i) + Xqn(j)*Yqz(i)); 
% 
%                 end
% 
%                 for k = (h-1)/2:-1:1
%                     i = k;
%                     j = h-i;  
%                     
%                     Zdz(h) = Zdz(h) + 0.5*(+Xdp(i)*Yqn(j)-Xqp(i)*Ydn(j)-Xdn(j)*Yqp(i)+Xqn(j)*Ydp(i));
%                     Zqz(h) = Zqz(h) + 0.5*(+Xdp(i)*Ydn(j)+Xqp(i)*Yqn(j)+Xdn(j)*Ydp(i)+Xqn(j)*Yqp(i));
%                     Zdz(h) = Zdz(h) + 0.5*(+Xdp(j)*Yqn(i)-Xqp(j)*Ydn(i)-Xdn(i)*Yqp(j)+Xqn(i)*Ydp(j));
%                     Zqz(h) = Zqz(h) + 0.5*(+Xdp(j)*Ydn(i)+Xqp(j)*Yqn(i)+Xdn(i)*Ydp(j)+Xqn(i)*Yqp(j)); 
%                     Zdz(h) = Zdz(h) + 0.5*(+Xdz(i)*Yqz(j)+Xqz(i)*Ydz(j)+Xdz(j)*Yqz(i)+Xqz(j)*Ydz(i));
%                     Zqz(h) = Zqz(h) + 0.5*(-Xdz(i)*Ydz(j)+Xqz(i)*Yqz(j)-Xdz(j)*Ydz(i)+Xqz(j)*Yqz(i));    
%                         
%                         
%                     Zdp(h) = Zdp(h) + 0.5*(+Xdz(i)*Yqp(j)+Xqz(i)*Ydp(j)+Xdz(j)*Yqp(i)+Xqz(j)*Ydp(i));
%                     Zqp(h) = Zqp(h) + 0.5*(-Xdz(i)*Ydp(j)+Xqz(i)*Yqp(j)-Xdz(j)*Ydp(i)+Xqz(j)*Yqp(i));
%                     Zdp(h) = Zdp(h) + 0.5*(+Xdp(i)*Yqz(j)+Xqp(i)*Ydz(j)+Xdp(j)*Yqz(i)+Xqp(j)*Ydz(i));
%                     Zqp(h) = Zqp(h) + 0.5*(-Xdp(i)*Ydz(j)+Xqp(i)*Yqz(j)-Xdp(j)*Ydz(i)+Xqp(j)*Yqz(i)); 
%                     
%                               
%                     Zdn(h) = Zdn(h) + 0.5*(+Xdn(i)*Yqz(j)-Xqn(i)*Ydz(j)+Xdn(j)*Yqz(i)-Xqn(j)*Ydz(i));
%                     Zqn(h) = Zqn(h) + 0.5*(+Xdn(i)*Ydz(j)+Xqn(i)*Yqz(j)+Xdn(j)*Ydz(i)+Xqn(j)*Yqz(i)); 
%                     Zdn(h) = Zdn(h) + 0.5*(-Xdz(i)*Yqn(j)+Xqz(i)*Ydn(j)-Xdz(j)*Yqn(i)+Xqz(j)*Ydn(i));
%                     Zqn(h) = Zqn(h) + 0.5*(+Xdz(i)*Ydn(j)+Xqz(i)*Yqn(j)+Xdz(j)*Ydn(i)+Xqz(j)*Yqn(i)); 
%                 end
% %%%%%%%%%%%%%%%%%%%%%% h<=N EVEN %%%%%%%%%%%%%%%%%%%%%%%%%%%%%%%%%%%%%%%%%           
%             else 
% 
%                 if(h <= N)                   
%                     Zdp(h) = Zdp(h) + 0.5*(-Xdn(h/2)*Yqn(h/2)-Xqn(h/2)*Ydn(h/2));   
%                     Zqp(h) = Zqp(h) + 0.5*(-Xdn(h/2)*Ydn(h/2)+Xqn(h/2)*Yqn(h/2)); 
%                     Zdn(h) = Zdn(h) + 0.5*(-Xdp(h/2)*Yqp(h/2)-Xqp(h/2)*Ydp(h/2));   
%                     Zqn(h) = Zqn(h) + 0.5*(-Xdp(h/2)*Ydp(h/2)+Xqp(h/2)*Yqp(h/2));   
% 
%                     Zdz(h)  = Zdz(h)  + 0.5*(+Xdz(h/2)*Yqz(h/2)+Xqz(h/2)*Ydz(h/2));
%                     Zqz(h)  = Zqz(h)  + 0.5*(-Xdz(h/2)*Ydz(h/2)+Xqz(h/2)*Yqz(h/2));
% 
%                     Zdp(h) = Zdp(h) + 0.5*(+Xdz(h/2)*Yqp(h/2)+Xqz(h/2)*Ydp(h/2)+Xdp(h/2)*Yqz(h/2)+Xqp(h/2)*Ydz(h/2));   
%                     Zqp(h) = Zqp(h) + 0.5*(-Xdz(h/2)*Ydp(h/2)+Xqz(h/2)*Yqp(h/2)-Xdp(h/2)*Ydz(h/2)+Xqp(h/2)*Yqz(h/2)); 
%                     Zdn(h) = Zdn(h) + 0.5*(+Xdn(h/2)*Yqz(h/2)-Xqn(h/2)*Ydz(h/2)-Xdz(h/2)*Yqn(h/2)+Xqz(h/2)*Ydn(h/2));   
%                     Zqn(h) = Zqn(h) + 0.5*(+Xdn(h/2)*Ydz(h/2)+Xqn(h/2)*Yqz(h/2)+Xdz(h/2)*Ydn(h/2)+Xqz(h/2)*Yqn(h/2));    
%                 end
%                 
%                 for k = 1:N-h
%                     i = k;
%                     j = h+i;
%                 
%                     Zdz(h) = Zdz(h)   + 0.5*(+Xdp(j)*Yqp(i) - Xqp(j)*Ydp(i) - Xdp(i)*Yqp(j) + Xqp(i)*Ydp(j));
%                     Zqz(h) = Zqz(h)   + 0.5*(+Xdp(j)*Ydp(i) + Xqp(j)*Yqp(i) + Xdp(i)*Ydp(j) + Xqp(i)*Yqp(j));                                           
%                     Zdz(h) = Zdz(h)   + 0.5*(+Xdn(i)*Yqn(j) - Xqn(i)*Ydn(j) - Xdn(j)*Yqn(i) + Xqn(j)*Ydn(i));
%                     Zqz(h) = Zqz(h)   + 0.5*(+Xdn(i)*Ydn(j) + Xqn(i)*Yqn(j) + Xdn(j)*Ydn(i) + Xqn(j)*Yqn(i));  
%                     Zdz(h) = Zdz(h)   + 0.5*(-Xdz(i)*Yqz(j) + Xqz(i)*Ydz(j) + Xdz(j)*Yqz(i) - Xqz(j)*Ydz(i));
%                     Zqz(h) = Zqz(h)   + 0.5*(+Xdz(i)*Ydz(j) + Xqz(i)*Yqz(j) + Xdz(j)*Ydz(i) + Xqz(j)*Yqz(i)); 
%                                        
%                     Zdp(h) = Zdp(h) + 0.5*(-Xdp(i)*Yqn(j) - Xqp(i)*Ydn(j) - Xdn(j)*Yqp(i) - Xqn(j)*Ydp(i)); 
%                     Zqp(h) = Zqp(h) + 0.5*(-Xdp(i)*Ydn(j) + Xqp(i)*Yqn(j) - Xdn(j)*Ydp(i) + Xqn(j)*Yqp(i)); 
%                     Zdn(h) = Zdn(h) + 0.5*(-Xdn(i)*Yqp(j) - Xqn(i)*Ydp(j) - Xdp(j)*Yqn(i) - Xqp(j)*Ydn(i)); 
%                     Zqn(h) = Zqn(h) + 0.5*(-Xdn(i)*Ydp(j) + Xqn(i)*Yqp(j) - Xdp(j)*Ydn(i) + Xqp(j)*Yqn(i)); 
%                         
%                     Zdp(h) = Zdp(h) + 0.5*(+Xdp(j)*Yqz(i) - Xqp(j)*Ydz(i) - Xdz(i)*Yqp(j) + Xqz(i)*Ydp(j));
%                     Zqp(h) = Zqp(h) + 0.5*(+Xdp(j)*Ydz(i) + Xqp(j)*Yqz(i) + Xdz(i)*Ydp(j) + Xqz(i)*Yqp(j)); 
%                     Zdn(h) = Zdn(h) + 0.5*(+Xdp(i)*Yqz(j) - Xqp(i)*Ydz(j) - Xdz(j)*Yqp(i) + Xqz(j)*Ydp(i));
%                     Zqn(h) = Zqn(h) + 0.5*(+Xdp(i)*Ydz(j) + Xqp(i)*Yqz(j) + Xdz(j)*Ydp(i) + Xqz(j)*Yqp(i)); 
%                     
%                     Zdp(h) = Zdp(h) + 0.5*(+Xdn(i)*Yqz(j) + Xqn(i)*Ydz(j) + Xdz(j)*Yqn(i) + Xqz(j)*Ydn(i));
%                     Zqp(h) = Zqp(h) + 0.5*(-Xdn(i)*Ydz(j) + Xqn(i)*Yqz(j) - Xdz(j)*Ydn(i) + Xqz(j)*Yqn(i)); 
%                     Zdn(h) = Zdn(h) + 0.5*(+Xdn(j)*Yqz(i) + Xqn(j)*Ydz(i) + Xdz(i)*Yqn(j) + Xqz(i)*Ydn(j));
%                     Zqn(h) = Zqn(h) + 0.5*(-Xdn(j)*Ydz(i) + Xqn(j)*Yqz(i) - Xdz(i)*Ydn(j) + Xqz(i)*Yqn(j)); 
%                 end
% 
%                 for k = h/2-1:-1:1
%                     i = k;
%                     j = h-i;   
% 
%                     Zdz(h) = Zdz(h)   + 0.5*(+Xdp(i)*Yqn(j) - Xqp(i)*Ydn(j) + Xdp(j)*Yqn(i) - Xqp(j)*Ydn(i));
%                     Zdz(h) = Zdz(h)   + 0.5*(-Xdn(i)*Yqp(j) + Xqn(i)*Ydp(j) - Xdn(j)*Yqp(i) + Xqn(j)*Ydp(i));      
%                     Zdz(h) = Zdz(h)   + 0.5*(+Xdz(i)*Yqz(j) + Xqz(i)*Ydz(j) + Xdz(j)*Yqz(i) + Xqz(j)*Ydz(i));
%                     
%                     Zqz(h) = Zqz(h)   + 0.5*(+Xdp(i)*Ydn(j) + Xqp(i)*Yqn(j) + Xdp(j)*Ydn(i) + Xqp(j)*Yqn(i)); 
%                     Zqz(h) = Zqz(h)   + 0.5*(+Xdn(i)*Ydp(j) + Xqn(i)*Yqp(j) + Xdn(j)*Ydp(i) + Xqn(j)*Yqp(i));
%                     Zqz(h) = Zqz(h)   + 0.5*(-Xdz(i)*Ydz(j) + Xqz(i)*Yqz(j) - Xdz(j)*Ydz(i) + Xqz(j)*Yqz(i)); 
%                     
%                     Zdp(h) = Zdp(h) + 0.5*(+Xdp(i)*Yqz(j) + Xqp(i)*Ydz(j) + Xdp(j)*Yqz(i) + Xqp(j)*Ydz(i)); 
%                     Zdp(h) = Zdp(h) + 0.5*(-Xdn(i)*Yqn(j) - Xqn(i)*Ydn(j) - Xdn(j)*Yqn(i) - Xqn(j)*Ydn(i)); 
%                     Zdp(h) = Zdp(h) + 0.5*(+Xdz(i)*Yqp(j) + Xqz(i)*Ydp(j) + Xdz(j)*Yqp(i) + Xqz(j)*Ydp(i));
%                     
%                     Zqp(h) = Zqp(h) + 0.5*(-Xdp(i)*Ydz(j) + Xqp(i)*Yqz(j) - Xdp(j)*Ydz(i) + Xqp(j)*Yqz(i)); 
%                     Zqp(h) = Zqp(h) + 0.5*(-Xdn(i)*Ydn(j) + Xqn(i)*Yqn(j) - Xdn(j)*Ydn(i) + Xqn(j)*Yqn(i));
%                     Zqp(h) = Zqp(h) + 0.5*(-Xdz(i)*Ydp(j) + Xqz(i)*Yqp(j) - Xdz(j)*Ydp(i) + Xqz(j)*Yqp(i));  
%                     
%                     Zdn(h) = Zdn(h) + 0.5*(-Xdp(i)*Yqp(j) - Xqp(i)*Ydp(j) - Xdp(j)*Yqp(i) - Xqp(j)*Ydp(i));
%                     Zdn(h) = Zdn(h) + 0.5*(+Xdn(i)*Yqz(j) - Xqn(i)*Ydz(j) + Xdn(j)*Yqz(i) - Xqn(j)*Ydz(i));
%                     Zdn(h) = Zdn(h) + 0.5*(-Xdz(i)*Yqn(j) + Xqz(i)*Ydn(j) - Xdz(j)*Yqn(i) + Xqz(j)*Ydn(i));
%                     
%                     Zqn(h) = Zqn(h) + 0.5*(-Xdp(i)*Ydp(j) + Xqp(i)*Yqp(j) - Xdp(j)*Ydp(i) + Xqp(j)*Yqp(i));  
%                     Zqn(h) = Zqn(h) + 0.5*(+Xdn(i)*Ydz(j) + Xqn(i)*Yqz(j) + Xdn(j)*Ydz(i) + Xqn(j)*Yqz(i));
%                     Zqn(h) = Zqn(h) + 0.5*(+Xdz(i)*Ydn(j) + Xqz(i)*Yqn(j) + Xdz(j)*Ydn(i) + Xqz(j)*Yqn(i)); 
%                 end
%             end
% %%%%%%%%%%%%%%%%%%%%%%%%%%%% h>N  %%%%%%%%%%%%%%%%%%%%%%%%%%%%%%%%%%%%%%%%% 
%         else %h>N
%             
%             
%             %%%%%%%%%%%%%%%%%%%%%%%%%%% PP + NN %%%%%%%%%%%%%%%%%%%%%%%%%%%
%             for i = h-N : N
%                 Zdp(h) = Zdp(h) - 0.5*(Xdn(i)*Yqn(h-i) + Xqn(i)*Ydn(h-i));                
%                 Zdn(h) = Zdn(h) - 0.5*(Xdp(i)*Yqp(h-i) + Xqp(i)*Ydp(h-i));                     
%                 Zqp(h) = Zqp(h) - 0.5*(Xdn(i)*Ydn(h-i) - Xqn(i)*Yqn(h-i));                      
%                 Zqn(h) = Zqn(h) - 0.5*(Xdp(i)*Ydp(h-i) - Xqp(i)*Yqp(h-i));   
%             end
%             %%%%%%%%%%%%%%%%%%%%%%%%%%% PP + NN %%%%%%%%%%%%%%%%%%%%%%%%%%%
% 
%             if(mod(h,2)==1) %%%%%%%%%%% h>N ODD %%%%%%%%%%%%%%%%%%%
% 
%                 for k = (h-1)/2:-1:h-N
%                     i = k;
%                     j = h-i;
%                     
%                     Zdz(h) = Zdz(h) + 0.5*(+Xdp(i)*Yqn(j)-Xqp(i)*Ydn(j)-Xdn(j)*Yqp(i)+Xqn(j)*Ydp(i));                  
%                     Zdz(h) = Zdz(h) + 0.5*(+Xdp(j)*Yqn(i)-Xqp(j)*Ydn(i)-Xdn(i)*Yqp(j)+Xqn(i)*Ydp(j));
%                     Zdz(h) = Zdz(h) + 0.5*(+Xdz(i)*Yqz(j)+Xqz(i)*Ydz(j)+Xdz(j)*Yqz(i)+Xqz(j)*Ydz(i));
%                     
%                     Zqz(h) = Zqz(h) + 0.5*(-Xdz(i)*Ydz(j)+Xqz(i)*Yqz(j)-Xdz(j)*Ydz(i)+Xqz(j)*Yqz(i));
%                     Zqz(h) = Zqz(h) + 0.5*(+Xdp(i)*Ydn(j)+Xqp(i)*Yqn(j)+Xdn(j)*Ydp(i)+Xqn(j)*Yqp(i));
%                     Zqz(h) = Zqz(h) + 0.5*(+Xdp(j)*Ydn(i)+Xqp(j)*Yqn(i)+Xdn(i)*Ydp(j)+Xqn(i)*Yqp(j));  
%                     
%                     Zdp(h) = Zdp(h) + 0.5*(+Xdp(i)*Yqz(j)+Xqp(i)*Ydz(j)+Xdp(j)*Yqz(i)+Xqp(j)*Ydz(i));
%                     Zdp(h) = Zdp(h) + 0.5*(+Xdz(i)*Yqp(j)+Xqz(i)*Ydp(j)+Xdz(j)*Yqp(i)+Xqz(j)*Ydp(i));
%                     
%                     Zqp(h) = Zqp(h) + 0.5*(-Xdp(i)*Ydz(j)+Xqp(i)*Yqz(j)-Xdp(j)*Ydz(i)+Xqp(j)*Yqz(i)); 
%                     Zqp(h) = Zqp(h) + 0.5*(-Xdz(i)*Ydp(j)+Xqz(i)*Yqp(j)-Xdz(j)*Ydp(i)+Xqz(j)*Yqp(i));     
%                                        
%                     Zdn(h) = Zdn(h) + 0.5*(+Xdn(i)*Yqz(j)-Xqn(i)*Ydz(j)+Xdn(j)*Yqz(i)-Xqn(j)*Ydz(i));
%                     Zdn(h) = Zdn(h) + 0.5*(-Xdz(i)*Yqn(j)+Xqz(i)*Ydn(j)-Xdz(j)*Yqn(i)+Xqz(j)*Ydn(i));
%                     
%                     Zqn(h) = Zqn(h) + 0.5*(+Xdn(i)*Ydz(j)+Xqn(i)*Yqz(j)+Xdn(j)*Ydz(i)+Xqn(j)*Yqz(i));
%                     Zqn(h) = Zqn(h) + 0.5*(+Xdz(i)*Ydn(j)+Xqz(i)*Yqn(j)+Xdz(j)*Ydn(i)+Xqz(j)*Yqn(i));    
% 
%                 end
% 
%             else %%%%%%%%%%% h>N EVEN %%%%%%%%%%%%%%%%%%%
% 
%                 Zdz(h)  = Zdz(h)  + 0.5*(+Xdz(h/2)*Yqz(h/2)+Xqz(h/2)*Ydz(h/2));
%                 Zqz(h)  = Zqz(h)  + 0.5*(-Xdz(h/2)*Ydz(h/2)+Xqz(h/2)*Yqz(h/2));
%                 
%                 Zdp(h) = 0.5*(-Xdn(h/2)*Yqn(h/2)-Xqn(h/2)*Ydn(h/2));          
%                 Zdp(h) = Zdp(h) + 0.5*(+Xdp(h/2)*Yqz(h/2)+Xqp(h/2)*Ydz(h/2));                
%                 Zdp(h) = Zdp(h) + 0.5*(+Xdz(h/2)*Yqp(h/2)+Xqz(h/2)*Ydp(h/2));    
%                 
%                 Zqp(h) = 0.5*(-Xdn(h/2)*Ydn(h/2)+Xqn(h/2)*Yqn(h/2));             
%                 Zqp(h) = Zqp(h) + 0.5*(-Xdp(h/2)*Ydz(h/2)+Xqp(h/2)*Yqz(h/2));        
%                 Zqp(h) = Zqp(h) + 0.5*(-Xdz(h/2)*Ydp(h/2)+Xqz(h/2)*Yqp(h/2)); 
%                 
%                 Zdn(h) = 0.5*(-Xdp(h/2)*Yqp(h/2)-Xqp(h/2)*Ydp(h/2)); 
%                 Zdn(h) = Zdn(h) + 0.5*(+Xdn(h/2)*Yqz(h/2)-Xqn(h/2)*Ydz(h/2));
%                 Zdn(h) = Zdn(h) + 0.5*(-Xdz(h/2)*Yqn(h/2)+Xqz(h/2)*Ydn(h/2));
%                                
%                 Zqn(h) = 0.5*(-Xdp(h/2)*Ydp(h/2)+Xqp(h/2)*Yqp(h/2)); 
%                 Zqn(h) = Zqn(h) + 0.5*(+Xdn(h/2)*Ydz(h/2)+Xqn(h/2)*Yqz(h/2));        
%                 Zqn(h) = Zqn(h) + 0.5*(+Xdz(h/2)*Ydn(h/2)+Xqz(h/2)*Yqn(h/2)); 
% 
%                 for i = (h+2)/2:N
%                     j = h-i;
%                     Zdz(h)  = Zdz(h)  + 0.5*(+Xdp(i)*Yqn(j)-Xqp(i)*Ydn(j)+Xdp(j)*Yqn(i)-Xqp(j)*Ydn(i));
%                     Zdz(h)  = Zdz(h)  + 0.5*(-Xdn(i)*Yqp(j)+Xqn(i)*Ydp(j)-Xdn(j)*Yqp(i)+Xqn(j)*Ydp(i));
%                     Zdz(h)  = Zdz(h)  + 0.5*(+Xdz(i)*Yqz(j)+Xqz(i)*Ydz(j)+Xdz(j)*Yqz(i)+Xqz(j)*Ydz(i));
%                     
%                     Zqz(h)  = Zqz(h)  + 0.5*(+Xdp(i)*Ydn(j)+Xqp(i)*Yqn(j)+Xdp(j)*Ydn(i)+Xqp(j)*Yqn(i));                      
%                     Zqz(h)  = Zqz(h)  + 0.5*(+Xdn(i)*Ydp(j)+Xqn(i)*Yqp(j)+Xdn(j)*Ydp(i)+Xqn(j)*Yqp(i));  
%                     Zqz(h)  = Zqz(h)  + 0.5*(-Xdz(i)*Ydz(j)+Xqz(i)*Yqz(j)-Xdz(j)*Ydz(i)+Xqz(j)*Yqz(i));
%                     
%                     Zdp(h) = Zdp(h) + 0.5*(+Xdp(i)*Yqz(j)+Xqp(i)*Ydz(j)+Xdp(j)*Yqz(i)+Xqp(j)*Ydz(i));  
%                     Zdp(h) = Zdp(h) + 0.5*(-Xdn(i)*Yqn(j)-Xqn(i)*Ydn(j)-Xdn(j)*Yqn(i)-Xqn(j)*Ydn(i));             
%                     Zdp(h) = Zdp(h) + 0.5*(+Xdz(i)*Yqp(j)+Xqz(i)*Ydp(j)+Xdz(j)*Yqp(i)+Xqz(j)*Ydp(i));           
%                     
%                     Zqp(h) = Zqp(h) + 0.5*(-Xdp(i)*Ydz(j)+Xqp(i)*Yqz(j)-Xdp(j)*Ydz(i)+Xqp(j)*Yqz(i));
%                     Zqp(h) = Zqp(h) + 0.5*(-Xdn(i)*Ydn(j)+Xqn(i)*Yqn(j)-Xdn(j)*Ydn(i)+Xqn(j)*Yqn(i));    
%                     Zqp(h) = Zqp(h) + 0.5*(-Xdz(i)*Ydp(j)+Xqz(i)*Yqp(j)-Xdz(j)*Ydp(i)+Xqz(j)*Yqp(i));   
%                     
%                     Zdn(h) = Zdn(h) + 0.5*(-Xdp(i)*Yqp(j)-Xqp(i)*Ydp(j)-Xdp(j)*Yqp(i)-Xqp(j)*Ydp(i));
%                     Zdn(h) = Zdn(h) + 0.5*(+Xdn(i)*Yqz(j)-Xqn(i)*Ydz(j)+Xdn(j)*Yqz(i)-Xqn(j)*Ydz(i));
%                     Zdn(h) = Zdn(h) + 0.5*(-Xdz(i)*Yqn(j)+Xqz(i)*Ydn(j)-Xdz(j)*Yqn(i)+Xqz(j)*Ydn(i));              
%                     
%                     Zqn(h) = Zqn(h) + 0.5*(-Xdp(i)*Ydp(j)+Xqp(i)*Yqp(j)-Xdp(j)*Ydp(i)+Xqp(j)*Yqp(i));
%                     Zqn(h) = Zqn(h) + 0.5*(+Xdn(i)*Ydz(j)+Xqn(i)*Yqz(j)+Xdn(j)*Ydz(i)+Xqn(j)*Yqz(i)); 
%                     Zqn(h) = Zqn(h) + 0.5*(+Xdz(i)*Ydn(j)+Xqz(i)*Yqn(j)+Xdz(j)*Ydn(i)+Xqz(j)*Yqn(i));  
%                 end
%             end
%         end  
%     end
% end
%     
%
